simulink model "AGL_FullLoop_DIAM4100"  (R2023a)
settings: Solver=FixedStepAuto  StartTime=0.0  StopTime=DIAM4100.validation.simTime_s  RelTol=1e-3
values from neighbouring files (symbols this model uses):
  DIAM4100 = evalin('base', 'DIAM4100')    [FullLoop_prepareDIAM4100.m]    (also in FullLoop_smokeTest.m)
  FullLoop = evalin('base', 'FullLoop')    [FullLoop_openModel.m]    (also in FullLoop_prepareDIAM4100.m; FullLoop_simParams.m = struct(); FullLoop_smokeTest.m)
undefined symbols (not defined in the file or in its folder): D1, lagging, pulse
libraries: spsSeriesRLCBranchLib x51, spsSaturableTransformerLib x51, spsPiSectionLineLib x50, spsCurrentMeasurementLib x9, spsThyristorLib x2, spsVoltageMeasurementLib x2, spsACVoltageSourceLib x1, slpidlib x1, spsLinearTransformerLib x1, spsPLLLib x1, spsPulseGeneratorThyristor6PulseLib x1, spsRMSLib x1
(part 1 of 2)
settings Model: Creator=KSSS  LastModifiedBy=KSSS

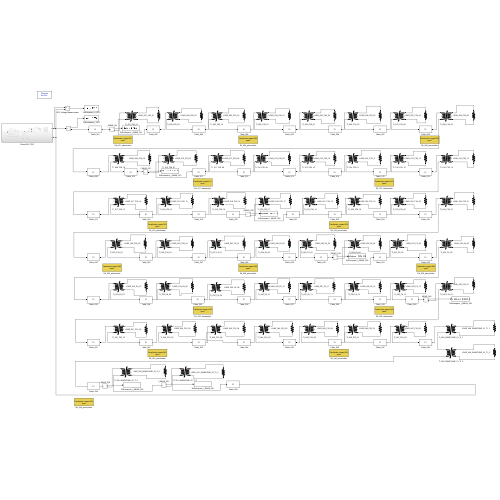
[thumbnail: Simulink's stored preview of the top-level diagram]
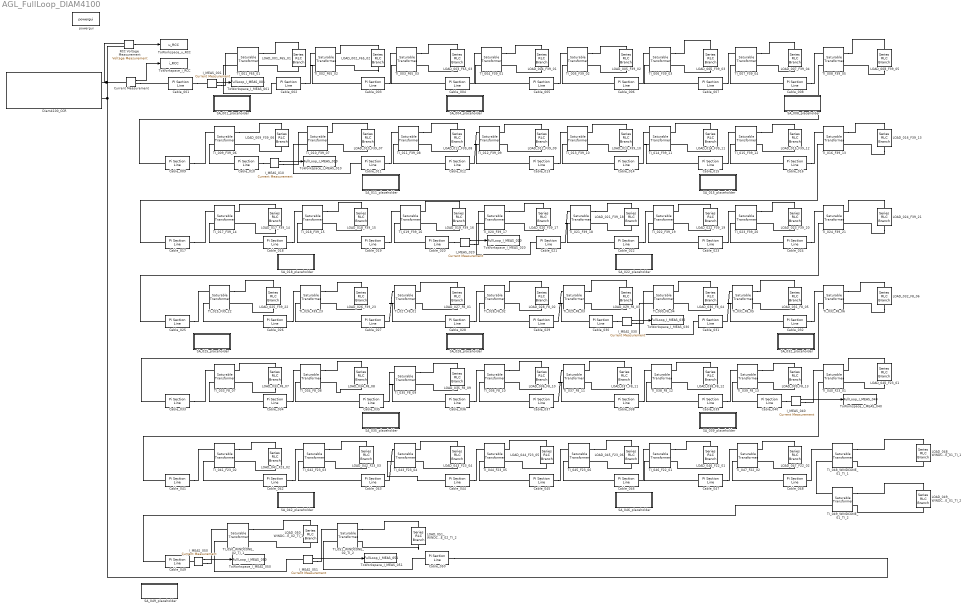
== system AGL_FullLoop_DIAM4100 ==
  Cable_001 : spsPiSectionLineLib/Pi Section Line  LConnTagsString=1  RConnTagsString=1  Phases=1  PiSections=1  Length=FullLoop.segments.length_km(1)  Frequency=FullLoop.grid.f_Hz  Resistance=FullLoop.cable.R_ohm_per_km  Inductance=FullLoop.cable.L_H_per_km  Capacitance=FullLoop.cable.C_F_per_km  SpecifyConductance=off  Conductance=0  Measurements=None  Measurements2=None
      settings: LibrarySourceBlock=sps_lib/Power Grid Elements/Pi Section Line
  Cable_002 : spsPiSectionLineLib/Pi Section Line  LConnTagsString=1  RConnTagsString=1  Phases=1  PiSections=1  Length=FullLoop.segments.length_km(2)  Frequency=FullLoop.grid.f_Hz  Resistance=FullLoop.cable.R_ohm_per_km  Inductance=FullLoop.cable.L_H_per_km  Capacitance=FullLoop.cable.C_F_per_km  SpecifyConductance=off  Conductance=0  Measurements=None  Measurements2=None
      settings: LibrarySourceBlock=sps_lib/Power Grid Elements/Pi Section Line
  Cable_003 : spsPiSectionLineLib/Pi Section Line  LConnTagsString=1  RConnTagsString=1  Phases=1  PiSections=1  Length=FullLoop.segments.length_km(3)  Frequency=FullLoop.grid.f_Hz  Resistance=FullLoop.cable.R_ohm_per_km  Inductance=FullLoop.cable.L_H_per_km  Capacitance=FullLoop.cable.C_F_per_km  SpecifyConductance=off  Conductance=0  Measurements=None  Measurements2=None
      settings: LibrarySourceBlock=sps_lib/Power Grid Elements/Pi Section Line
  Cable_004 : spsPiSectionLineLib/Pi Section Line  LConnTagsString=1  RConnTagsString=1  Phases=1  PiSections=1  Length=FullLoop.segments.length_km(4)  Frequency=FullLoop.grid.f_Hz  Resistance=FullLoop.cable.R_ohm_per_km  Inductance=FullLoop.cable.L_H_per_km  Capacitance=FullLoop.cable.C_F_per_km  SpecifyConductance=off  Conductance=0  Measurements=None  Measurements2=None
      settings: LibrarySourceBlock=sps_lib/Power Grid Elements/Pi Section Line
  Cable_005 : spsPiSectionLineLib/Pi Section Line  LConnTagsString=1  RConnTagsString=1  Phases=1  PiSections=1  Length=FullLoop.segments.length_km(5)  Frequency=FullLoop.grid.f_Hz  Resistance=FullLoop.cable.R_ohm_per_km  Inductance=FullLoop.cable.L_H_per_km  Capacitance=FullLoop.cable.C_F_per_km  SpecifyConductance=off  Conductance=0  Measurements=None  Measurements2=None
      settings: LibrarySourceBlock=sps_lib/Power Grid Elements/Pi Section Line
  Cable_006 : spsPiSectionLineLib/Pi Section Line  LConnTagsString=1  RConnTagsString=1  Phases=1  PiSections=1  Length=FullLoop.segments.length_km(6)  Frequency=FullLoop.grid.f_Hz  Resistance=FullLoop.cable.R_ohm_per_km  Inductance=FullLoop.cable.L_H_per_km  Capacitance=FullLoop.cable.C_F_per_km  SpecifyConductance=off  Conductance=0  Measurements=None  Measurements2=None
      settings: LibrarySourceBlock=sps_lib/Power Grid Elements/Pi Section Line
  Cable_007 : spsPiSectionLineLib/Pi Section Line  LConnTagsString=1  RConnTagsString=1  Phases=1  PiSections=1  Length=FullLoop.segments.length_km(7)  Frequency=FullLoop.grid.f_Hz  Resistance=FullLoop.cable.R_ohm_per_km  Inductance=FullLoop.cable.L_H_per_km  Capacitance=FullLoop.cable.C_F_per_km  SpecifyConductance=off  Conductance=0  Measurements=None  Measurements2=None
      settings: LibrarySourceBlock=sps_lib/Power Grid Elements/Pi Section Line
  Cable_008 : spsPiSectionLineLib/Pi Section Line  LConnTagsString=1  RConnTagsString=1  Phases=1  PiSections=1  Length=FullLoop.segments.length_km(8)  Frequency=FullLoop.grid.f_Hz  Resistance=FullLoop.cable.R_ohm_per_km  Inductance=FullLoop.cable.L_H_per_km  Capacitance=FullLoop.cable.C_F_per_km  SpecifyConductance=off  Conductance=0  Measurements=None  Measurements2=None
      settings: LibrarySourceBlock=sps_lib/Power Grid Elements/Pi Section Line
  Cable_009 : spsPiSectionLineLib/Pi Section Line  LConnTagsString=1  RConnTagsString=1  Phases=1  PiSections=1  Length=FullLoop.segments.length_km(9)  Frequency=FullLoop.grid.f_Hz  Resistance=FullLoop.cable.R_ohm_per_km  Inductance=FullLoop.cable.L_H_per_km  Capacitance=FullLoop.cable.C_F_per_km  SpecifyConductance=off  Conductance=0  Measurements=None  Measurements2=None
      settings: LibrarySourceBlock=sps_lib/Power Grid Elements/Pi Section Line
  Cable_010 : spsPiSectionLineLib/Pi Section Line  LConnTagsString=1  RConnTagsString=1  Phases=1  PiSections=1  Length=FullLoop.segments.length_km(10)  Frequency=FullLoop.grid.f_Hz  Resistance=FullLoop.cable.R_ohm_per_km  Inductance=FullLoop.cable.L_H_per_km  Capacitance=FullLoop.cable.C_F_per_km  SpecifyConductance=off  Conductance=0  Measurements=None  Measurements2=None
      settings: LibrarySourceBlock=sps_lib/Power Grid Elements/Pi Section Line
  Cable_011 : spsPiSectionLineLib/Pi Section Line  LConnTagsString=1  RConnTagsString=1  Phases=1  PiSections=1  Length=FullLoop.segments.length_km(11)  Frequency=FullLoop.grid.f_Hz  Resistance=FullLoop.cable.R_ohm_per_km  Inductance=FullLoop.cable.L_H_per_km  Capacitance=FullLoop.cable.C_F_per_km  SpecifyConductance=off  Conductance=0  Measurements=None  Measurements2=None
      settings: LibrarySourceBlock=sps_lib/Power Grid Elements/Pi Section Line
  Cable_012 : spsPiSectionLineLib/Pi Section Line  LConnTagsString=1  RConnTagsString=1  Phases=1  PiSections=1  Length=FullLoop.segments.length_km(12)  Frequency=FullLoop.grid.f_Hz  Resistance=FullLoop.cable.R_ohm_per_km  Inductance=FullLoop.cable.L_H_per_km  Capacitance=FullLoop.cable.C_F_per_km  SpecifyConductance=off  Conductance=0  Measurements=None  Measurements2=None
      settings: LibrarySourceBlock=sps_lib/Power Grid Elements/Pi Section Line
  Cable_013 : spsPiSectionLineLib/Pi Section Line  LConnTagsString=1  RConnTagsString=1  Phases=1  PiSections=1  Length=FullLoop.segments.length_km(13)  Frequency=FullLoop.grid.f_Hz  Resistance=FullLoop.cable.R_ohm_per_km  Inductance=FullLoop.cable.L_H_per_km  Capacitance=FullLoop.cable.C_F_per_km  SpecifyConductance=off  Conductance=0  Measurements=None  Measurements2=None
      settings: LibrarySourceBlock=sps_lib/Power Grid Elements/Pi Section Line
  Cable_014 : spsPiSectionLineLib/Pi Section Line  LConnTagsString=1  RConnTagsString=1  Phases=1  PiSections=1  Length=FullLoop.segments.length_km(14)  Frequency=FullLoop.grid.f_Hz  Resistance=FullLoop.cable.R_ohm_per_km  Inductance=FullLoop.cable.L_H_per_km  Capacitance=FullLoop.cable.C_F_per_km  SpecifyConductance=off  Conductance=0  Measurements=None  Measurements2=None
      settings: LibrarySourceBlock=sps_lib/Power Grid Elements/Pi Section Line
  Cable_015 : spsPiSectionLineLib/Pi Section Line  LConnTagsString=1  RConnTagsString=1  Phases=1  PiSections=1  Length=FullLoop.segments.length_km(15)  Frequency=FullLoop.grid.f_Hz  Resistance=FullLoop.cable.R_ohm_per_km  Inductance=FullLoop.cable.L_H_per_km  Capacitance=FullLoop.cable.C_F_per_km  SpecifyConductance=off  Conductance=0  Measurements=None  Measurements2=None
      settings: LibrarySourceBlock=sps_lib/Power Grid Elements/Pi Section Line
  Cable_016 : spsPiSectionLineLib/Pi Section Line  LConnTagsString=1  RConnTagsString=1  Phases=1  PiSections=1  Length=FullLoop.segments.length_km(16)  Frequency=FullLoop.grid.f_Hz  Resistance=FullLoop.cable.R_ohm_per_km  Inductance=FullLoop.cable.L_H_per_km  Capacitance=FullLoop.cable.C_F_per_km  SpecifyConductance=off  Conductance=0  Measurements=None  Measurements2=None
      settings: LibrarySourceBlock=sps_lib/Power Grid Elements/Pi Section Line
  Cable_017 : spsPiSectionLineLib/Pi Section Line  LConnTagsString=1  RConnTagsString=1  Phases=1  PiSections=1  Length=FullLoop.segments.length_km(17)  Frequency=FullLoop.grid.f_Hz  Resistance=FullLoop.cable.R_ohm_per_km  Inductance=FullLoop.cable.L_H_per_km  Capacitance=FullLoop.cable.C_F_per_km  SpecifyConductance=off  Conductance=0  Measurements=None  Measurements2=None
      settings: LibrarySourceBlock=sps_lib/Power Grid Elements/Pi Section Line
  Cable_018 : spsPiSectionLineLib/Pi Section Line  LConnTagsString=1  RConnTagsString=1  Phases=1  PiSections=1  Length=FullLoop.segments.length_km(18)  Frequency=FullLoop.grid.f_Hz  Resistance=FullLoop.cable.R_ohm_per_km  Inductance=FullLoop.cable.L_H_per_km  Capacitance=FullLoop.cable.C_F_per_km  SpecifyConductance=off  Conductance=0  Measurements=None  Measurements2=None
      settings: LibrarySourceBlock=sps_lib/Power Grid Elements/Pi Section Line
  Cable_019 : spsPiSectionLineLib/Pi Section Line  LConnTagsString=1  RConnTagsString=1  Phases=1  PiSections=1  Length=FullLoop.segments.length_km(19)  Frequency=FullLoop.grid.f_Hz  Resistance=FullLoop.cable.R_ohm_per_km  Inductance=FullLoop.cable.L_H_per_km  Capacitance=FullLoop.cable.C_F_per_km  SpecifyConductance=off  Conductance=0  Measurements=None  Measurements2=None
      settings: LibrarySourceBlock=sps_lib/Power Grid Elements/Pi Section Line
  Cable_020 : spsPiSectionLineLib/Pi Section Line  LConnTagsString=1  RConnTagsString=1  Phases=1  PiSections=1  Length=FullLoop.segments.length_km(20)  Frequency=FullLoop.grid.f_Hz  Resistance=FullLoop.cable.R_ohm_per_km  Inductance=FullLoop.cable.L_H_per_km  Capacitance=FullLoop.cable.C_F_per_km  SpecifyConductance=off  Conductance=0  Measurements=None  Measurements2=None
      settings: LibrarySourceBlock=sps_lib/Power Grid Elements/Pi Section Line
  Cable_021 : spsPiSectionLineLib/Pi Section Line  LConnTagsString=1  RConnTagsString=1  Phases=1  PiSections=1  Length=FullLoop.segments.length_km(21)  Frequency=FullLoop.grid.f_Hz  Resistance=FullLoop.cable.R_ohm_per_km  Inductance=FullLoop.cable.L_H_per_km  Capacitance=FullLoop.cable.C_F_per_km  SpecifyConductance=off  Conductance=0  Measurements=None  Measurements2=None
      settings: LibrarySourceBlock=sps_lib/Power Grid Elements/Pi Section Line
  Cable_022 : spsPiSectionLineLib/Pi Section Line  LConnTagsString=1  RConnTagsString=1  Phases=1  PiSections=1  Length=FullLoop.segments.length_km(22)  Frequency=FullLoop.grid.f_Hz  Resistance=FullLoop.cable.R_ohm_per_km  Inductance=FullLoop.cable.L_H_per_km  Capacitance=FullLoop.cable.C_F_per_km  SpecifyConductance=off  Conductance=0  Measurements=None  Measurements2=None
      settings: LibrarySourceBlock=sps_lib/Power Grid Elements/Pi Section Line
  Cable_023 : spsPiSectionLineLib/Pi Section Line  LConnTagsString=1  RConnTagsString=1  Phases=1  PiSections=1  Length=FullLoop.segments.length_km(23)  Frequency=FullLoop.grid.f_Hz  Resistance=FullLoop.cable.R_ohm_per_km  Inductance=FullLoop.cable.L_H_per_km  Capacitance=FullLoop.cable.C_F_per_km  SpecifyConductance=off  Conductance=0  Measurements=None  Measurements2=None
      settings: LibrarySourceBlock=sps_lib/Power Grid Elements/Pi Section Line
  Cable_024 : spsPiSectionLineLib/Pi Section Line  LConnTagsString=1  RConnTagsString=1  Phases=1  PiSections=1  Length=FullLoop.segments.length_km(24)  Frequency=FullLoop.grid.f_Hz  Resistance=FullLoop.cable.R_ohm_per_km  Inductance=FullLoop.cable.L_H_per_km  Capacitance=FullLoop.cable.C_F_per_km  SpecifyConductance=off  Conductance=0  Measurements=None  Measurements2=None
      settings: LibrarySourceBlock=sps_lib/Power Grid Elements/Pi Section Line
  Cable_025 : spsPiSectionLineLib/Pi Section Line  LConnTagsString=1  RConnTagsString=1  Phases=1  PiSections=1  Length=FullLoop.segments.length_km(25)  Frequency=FullLoop.grid.f_Hz  Resistance=FullLoop.cable.R_ohm_per_km  Inductance=FullLoop.cable.L_H_per_km  Capacitance=FullLoop.cable.C_F_per_km  SpecifyConductance=off  Conductance=0  Measurements=None  Measurements2=None
      settings: LibrarySourceBlock=sps_lib/Power Grid Elements/Pi Section Line
  Cable_026 : spsPiSectionLineLib/Pi Section Line  LConnTagsString=1  RConnTagsString=1  Phases=1  PiSections=1  Length=FullLoop.segments.length_km(26)  Frequency=FullLoop.grid.f_Hz  Resistance=FullLoop.cable.R_ohm_per_km  Inductance=FullLoop.cable.L_H_per_km  Capacitance=FullLoop.cable.C_F_per_km  SpecifyConductance=off  Conductance=0  Measurements=None  Measurements2=None
      settings: LibrarySourceBlock=sps_lib/Power Grid Elements/Pi Section Line
  Cable_027 : spsPiSectionLineLib/Pi Section Line  LConnTagsString=1  RConnTagsString=1  Phases=1  PiSections=1  Length=FullLoop.segments.length_km(27)  Frequency=FullLoop.grid.f_Hz  Resistance=FullLoop.cable.R_ohm_per_km  Inductance=FullLoop.cable.L_H_per_km  Capacitance=FullLoop.cable.C_F_per_km  SpecifyConductance=off  Conductance=0  Measurements=None  Measurements2=None
      settings: LibrarySourceBlock=sps_lib/Power Grid Elements/Pi Section Line
  Cable_028 : spsPiSectionLineLib/Pi Section Line  LConnTagsString=1  RConnTagsString=1  Phases=1  PiSections=1  Length=FullLoop.segments.length_km(28)  Frequency=FullLoop.grid.f_Hz  Resistance=FullLoop.cable.R_ohm_per_km  Inductance=FullLoop.cable.L_H_per_km  Capacitance=FullLoop.cable.C_F_per_km  SpecifyConductance=off  Conductance=0  Measurements=None  Measurements2=None
      settings: LibrarySourceBlock=sps_lib/Power Grid Elements/Pi Section Line
  Cable_029 : spsPiSectionLineLib/Pi Section Line  LConnTagsString=1  RConnTagsString=1  Phases=1  PiSections=1  Length=FullLoop.segments.length_km(29)  Frequency=FullLoop.grid.f_Hz  Resistance=FullLoop.cable.R_ohm_per_km  Inductance=FullLoop.cable.L_H_per_km  Capacitance=FullLoop.cable.C_F_per_km  SpecifyConductance=off  Conductance=0  Measurements=None  Measurements2=None
      settings: LibrarySourceBlock=sps_lib/Power Grid Elements/Pi Section Line
  Cable_030 : spsPiSectionLineLib/Pi Section Line  LConnTagsString=1  RConnTagsString=1  Phases=1  PiSections=1  Length=FullLoop.segments.length_km(30)  Frequency=FullLoop.grid.f_Hz  Resistance=FullLoop.cable.R_ohm_per_km  Inductance=FullLoop.cable.L_H_per_km  Capacitance=FullLoop.cable.C_F_per_km  SpecifyConductance=off  Conductance=0  Measurements=None  Measurements2=None
      settings: LibrarySourceBlock=sps_lib/Power Grid Elements/Pi Section Line
  Cable_031 : spsPiSectionLineLib/Pi Section Line  LConnTagsString=1  RConnTagsString=1  Phases=1  PiSections=1  Length=FullLoop.segments.length_km(31)  Frequency=FullLoop.grid.f_Hz  Resistance=FullLoop.cable.R_ohm_per_km  Inductance=FullLoop.cable.L_H_per_km  Capacitance=FullLoop.cable.C_F_per_km  SpecifyConductance=off  Conductance=0  Measurements=None  Measurements2=None
      settings: LibrarySourceBlock=sps_lib/Power Grid Elements/Pi Section Line
  Cable_032 : spsPiSectionLineLib/Pi Section Line  LConnTagsString=1  RConnTagsString=1  Phases=1  PiSections=1  Length=FullLoop.segments.length_km(32)  Frequency=FullLoop.grid.f_Hz  Resistance=FullLoop.cable.R_ohm_per_km  Inductance=FullLoop.cable.L_H_per_km  Capacitance=FullLoop.cable.C_F_per_km  SpecifyConductance=off  Conductance=0  Measurements=None  Measurements2=None
      settings: LibrarySourceBlock=sps_lib/Power Grid Elements/Pi Section Line
  Cable_033 : spsPiSectionLineLib/Pi Section Line  LConnTagsString=1  RConnTagsString=1  Phases=1  PiSections=1  Length=FullLoop.segments.length_km(33)  Frequency=FullLoop.grid.f_Hz  Resistance=FullLoop.cable.R_ohm_per_km  Inductance=FullLoop.cable.L_H_per_km  Capacitance=FullLoop.cable.C_F_per_km  SpecifyConductance=off  Conductance=0  Measurements=None  Measurements2=None
      settings: LibrarySourceBlock=sps_lib/Power Grid Elements/Pi Section Line
  Cable_034 : spsPiSectionLineLib/Pi Section Line  LConnTagsString=1  RConnTagsString=1  Phases=1  PiSections=1  Length=FullLoop.segments.length_km(34)  Frequency=FullLoop.grid.f_Hz  Resistance=FullLoop.cable.R_ohm_per_km  Inductance=FullLoop.cable.L_H_per_km  Capacitance=FullLoop.cable.C_F_per_km  SpecifyConductance=off  Conductance=0  Measurements=None  Measurements2=None
      settings: LibrarySourceBlock=sps_lib/Power Grid Elements/Pi Section Line
  Cable_035 : spsPiSectionLineLib/Pi Section Line  LConnTagsString=1  RConnTagsString=1  Phases=1  PiSections=1  Length=FullLoop.segments.length_km(35)  Frequency=FullLoop.grid.f_Hz  Resistance=FullLoop.cable.R_ohm_per_km  Inductance=FullLoop.cable.L_H_per_km  Capacitance=FullLoop.cable.C_F_per_km  SpecifyConductance=off  Conductance=0  Measurements=None  Measurements2=None
      settings: LibrarySourceBlock=sps_lib/Power Grid Elements/Pi Section Line
  Cable_036 : spsPiSectionLineLib/Pi Section Line  LConnTagsString=1  RConnTagsString=1  Phases=1  PiSections=1  Length=FullLoop.segments.length_km(36)  Frequency=FullLoop.grid.f_Hz  Resistance=FullLoop.cable.R_ohm_per_km  Inductance=FullLoop.cable.L_H_per_km  Capacitance=FullLoop.cable.C_F_per_km  SpecifyConductance=off  Conductance=0  Measurements=None  Measurements2=None
      settings: LibrarySourceBlock=sps_lib/Power Grid Elements/Pi Section Line
  Cable_037 : spsPiSectionLineLib/Pi Section Line  LConnTagsString=1  RConnTagsString=1  Phases=1  PiSections=1  Length=FullLoop.segments.length_km(37)  Frequency=FullLoop.grid.f_Hz  Resistance=FullLoop.cable.R_ohm_per_km  Inductance=FullLoop.cable.L_H_per_km  Capacitance=FullLoop.cable.C_F_per_km  SpecifyConductance=off  Conductance=0  Measurements=None  Measurements2=None
      settings: LibrarySourceBlock=sps_lib/Power Grid Elements/Pi Section Line
  Cable_038 : spsPiSectionLineLib/Pi Section Line  LConnTagsString=1  RConnTagsString=1  Phases=1  PiSections=1  Length=FullLoop.segments.length_km(38)  Frequency=FullLoop.grid.f_Hz  Resistance=FullLoop.cable.R_ohm_per_km  Inductance=FullLoop.cable.L_H_per_km  Capacitance=FullLoop.cable.C_F_per_km  SpecifyConductance=off  Conductance=0  Measurements=None  Measurements2=None
      settings: LibrarySourceBlock=sps_lib/Power Grid Elements/Pi Section Line
  Cable_039 : spsPiSectionLineLib/Pi Section Line  LConnTagsString=1  RConnTagsString=1  Phases=1  PiSections=1  Length=FullLoop.segments.length_km(39)  Frequency=FullLoop.grid.f_Hz  Resistance=FullLoop.cable.R_ohm_per_km  Inductance=FullLoop.cable.L_H_per_km  Capacitance=FullLoop.cable.C_F_per_km  SpecifyConductance=off  Conductance=0  Measurements=None  Measurements2=None
      settings: LibrarySourceBlock=sps_lib/Power Grid Elements/Pi Section Line
  Cable_040 : spsPiSectionLineLib/Pi Section Line  LConnTagsString=1  RConnTagsString=1  Phases=1  PiSections=1  Length=FullLoop.segments.length_km(40)  Frequency=FullLoop.grid.f_Hz  Resistance=FullLoop.cable.R_ohm_per_km  Inductance=FullLoop.cable.L_H_per_km  Capacitance=FullLoop.cable.C_F_per_km  SpecifyConductance=off  Conductance=0  Measurements=None  Measurements2=None
      settings: LibrarySourceBlock=sps_lib/Power Grid Elements/Pi Section Line
  Cable_041 : spsPiSectionLineLib/Pi Section Line  LConnTagsString=1  RConnTagsString=1  Phases=1  PiSections=1  Length=FullLoop.segments.length_km(41)  Frequency=FullLoop.grid.f_Hz  Resistance=FullLoop.cable.R_ohm_per_km  Inductance=FullLoop.cable.L_H_per_km  Capacitance=FullLoop.cable.C_F_per_km  SpecifyConductance=off  Conductance=0  Measurements=None  Measurements2=None
      settings: LibrarySourceBlock=sps_lib/Power Grid Elements/Pi Section Line
  Cable_042 : spsPiSectionLineLib/Pi Section Line  LConnTagsString=1  RConnTagsString=1  Phases=1  PiSections=1  Length=FullLoop.segments.length_km(42)  Frequency=FullLoop.grid.f_Hz  Resistance=FullLoop.cable.R_ohm_per_km  Inductance=FullLoop.cable.L_H_per_km  Capacitance=FullLoop.cable.C_F_per_km  SpecifyConductance=off  Conductance=0  Measurements=None  Measurements2=None
      settings: LibrarySourceBlock=sps_lib/Power Grid Elements/Pi Section Line
  Cable_043 : spsPiSectionLineLib/Pi Section Line  LConnTagsString=1  RConnTagsString=1  Phases=1  PiSections=1  Length=FullLoop.segments.length_km(43)  Frequency=FullLoop.grid.f_Hz  Resistance=FullLoop.cable.R_ohm_per_km  Inductance=FullLoop.cable.L_H_per_km  Capacitance=FullLoop.cable.C_F_per_km  SpecifyConductance=off  Conductance=0  Measurements=None  Measurements2=None
      settings: LibrarySourceBlock=sps_lib/Power Grid Elements/Pi Section Line
  Cable_044 : spsPiSectionLineLib/Pi Section Line  LConnTagsString=1  RConnTagsString=1  Phases=1  PiSections=1  Length=FullLoop.segments.length_km(44)  Frequency=FullLoop.grid.f_Hz  Resistance=FullLoop.cable.R_ohm_per_km  Inductance=FullLoop.cable.L_H_per_km  Capacitance=FullLoop.cable.C_F_per_km  SpecifyConductance=off  Conductance=0  Measurements=None  Measurements2=None
      settings: LibrarySourceBlock=sps_lib/Power Grid Elements/Pi Section Line
  Cable_045 : spsPiSectionLineLib/Pi Section Line  LConnTagsString=1  RConnTagsString=1  Phases=1  PiSections=1  Length=FullLoop.segments.length_km(45)  Frequency=FullLoop.grid.f_Hz  Resistance=FullLoop.cable.R_ohm_per_km  Inductance=FullLoop.cable.L_H_per_km  Capacitance=FullLoop.cable.C_F_per_km  SpecifyConductance=off  Conductance=0  Measurements=None  Measurements2=None
      settings: LibrarySourceBlock=sps_lib/Power Grid Elements/Pi Section Line
  Cable_046 : spsPiSectionLineLib/Pi Section Line  LConnTagsString=1  RConnTagsString=1  Phases=1  PiSections=1  Length=FullLoop.segments.length_km(46)  Frequency=FullLoop.grid.f_Hz  Resistance=FullLoop.cable.R_ohm_per_km  Inductance=FullLoop.cable.L_H_per_km  Capacitance=FullLoop.cable.C_F_per_km  SpecifyConductance=off  Conductance=0  Measurements=None  Measurements2=None
      settings: LibrarySourceBlock=sps_lib/Power Grid Elements/Pi Section Line
  Cable_047 : spsPiSectionLineLib/Pi Section Line  LConnTagsString=1  RConnTagsString=1  Phases=1  PiSections=1  Length=FullLoop.segments.length_km(47)  Frequency=FullLoop.grid.f_Hz  Resistance=FullLoop.cable.R_ohm_per_km  Inductance=FullLoop.cable.L_H_per_km  Capacitance=FullLoop.cable.C_F_per_km  SpecifyConductance=off  Conductance=0  Measurements=None  Measurements2=None
      settings: LibrarySourceBlock=sps_lib/Power Grid Elements/Pi Section Line
  Cable_048 : spsPiSectionLineLib/Pi Section Line  LConnTagsString=1  RConnTagsString=1  Phases=1  PiSections=1  Length=FullLoop.segments.length_km(48)  Frequency=FullLoop.grid.f_Hz  Resistance=FullLoop.cable.R_ohm_per_km  Inductance=FullLoop.cable.L_H_per_km  Capacitance=FullLoop.cable.C_F_per_km  SpecifyConductance=off  Conductance=0  Measurements=None  Measurements2=None
      settings: LibrarySourceBlock=sps_lib/Power Grid Elements/Pi Section Line
  Cable_049 : spsPiSectionLineLib/Pi Section Line  LConnTagsString=1  RConnTagsString=1  Phases=1  PiSections=1  Length=FullLoop.segments.length_km(49)  Frequency=FullLoop.grid.f_Hz  Resistance=FullLoop.cable.R_ohm_per_km  Inductance=FullLoop.cable.L_H_per_km  Capacitance=FullLoop.cable.C_F_per_km  SpecifyConductance=off  Conductance=0  Measurements=None  Measurements2=None
      settings: LibrarySourceBlock=sps_lib/Power Grid Elements/Pi Section Line
  Cable_050 : spsPiSectionLineLib/Pi Section Line  LConnTagsString=1  RConnTagsString=1  Phases=1  PiSections=1  Length=FullLoop.segments.length_km(50)  Frequency=FullLoop.grid.f_Hz  Resistance=FullLoop.cable.R_ohm_per_km  Inductance=FullLoop.cable.L_H_per_km  Capacitance=FullLoop.cable.C_F_per_km  SpecifyConductance=off  Conductance=0  Measurements=None  Measurements2=None
      settings: LibrarySourceBlock=sps_lib/Power Grid Elements/Pi Section Line
  Current Measurement : spsCurrentMeasurementLib/Current Measurement  PhasorSimulation=off  OutputType=Complex  PSBequivalent=0
  Diam4100_CCR : Subsystem
  I_MEAS_001 : spsCurrentMeasurementLib/Current Measurement  PhasorSimulation=off  OutputType=Complex  PSBequivalent=0
  I_MEAS_010 : spsCurrentMeasurementLib/Current Measurement  PhasorSimulation=off  OutputType=Complex  PSBequivalent=0
  I_MEAS_020 : spsCurrentMeasurementLib/Current Measurement  PhasorSimulation=off  OutputType=Complex  PSBequivalent=0
  I_MEAS_030 : spsCurrentMeasurementLib/Current Measurement  PhasorSimulation=off  OutputType=Complex  PSBequivalent=0
  I_MEAS_040 : spsCurrentMeasurementLib/Current Measurement  PhasorSimulation=off  OutputType=Complex  PSBequivalent=0
  I_MEAS_050 : spsCurrentMeasurementLib/Current Measurement  PhasorSimulation=off  OutputType=Complex  PSBequivalent=0
  I_MEAS_051 : spsCurrentMeasurementLib/Current Measurement  PhasorSimulation=off  OutputType=Complex  PSBequivalent=0
  LOAD_001_F65_01 : spsSeriesRLCBranchLib/Series RLC Branch  LConnTagsString=__new0  RConnTagsString=__new0  BranchType=R  Resistance=FullLoop.loads(1).SecondaryResistance_ohm  Inductance=1e-3  SetiL0=off  InitialCurrent=0  Capacitance=1e-6  Setx0=off  InitialVoltage=0  Measurements=None
  LOAD_002_F65_02 : spsSeriesRLCBranchLib/Series RLC Branch  LConnTagsString=__new0  RConnTagsString=__new0  BranchType=R  Resistance=FullLoop.loads(2).SecondaryResistance_ohm  Inductance=1e-3  SetiL0=off  InitialCurrent=0  Capacitance=1e-6  Setx0=off  InitialVoltage=0  Measurements=None
  LOAD_003_F65_03 : spsSeriesRLCBranchLib/Series RLC Branch  LConnTagsString=__new0  RConnTagsString=__new0  BranchType=R  Resistance=FullLoop.loads(3).SecondaryResistance_ohm  Inductance=1e-3  SetiL0=off  InitialCurrent=0  Capacitance=1e-6  Setx0=off  InitialVoltage=0  Measurements=None
  LOAD_004_F39_01 : spsSeriesRLCBranchLib/Series RLC Branch  LConnTagsString=__new0  RConnTagsString=__new0  BranchType=R  Resistance=FullLoop.loads(4).SecondaryResistance_ohm  Inductance=1e-3  SetiL0=off  InitialCurrent=0  Capacitance=1e-6  Setx0=off  InitialVoltage=0  Measurements=None
  LOAD_005_F39_02 : spsSeriesRLCBranchLib/Series RLC Branch  LConnTagsString=__new0  RConnTagsString=__new0  BranchType=R  Resistance=FullLoop.loads(5).SecondaryResistance_ohm  Inductance=1e-3  SetiL0=off  InitialCurrent=0  Capacitance=1e-6  Setx0=off  InitialVoltage=0  Measurements=None
  LOAD_006_F39_03 : spsSeriesRLCBranchLib/Series RLC Branch  LConnTagsString=__new0  RConnTagsString=__new0  BranchType=R  Resistance=FullLoop.loads(6).SecondaryResistance_ohm  Inductance=1e-3  SetiL0=off  InitialCurrent=0  Capacitance=1e-6  Setx0=off  InitialVoltage=0  Measurements=None
  LOAD_007_F39_04 : spsSeriesRLCBranchLib/Series RLC Branch  LConnTagsString=__new0  RConnTagsString=__new0  BranchType=R  Resistance=FullLoop.loads(7).SecondaryResistance_ohm  Inductance=1e-3  SetiL0=off  InitialCurrent=0  Capacitance=1e-6  Setx0=off  InitialVoltage=0  Measurements=None
  LOAD_008_F39_05 : spsSeriesRLCBranchLib/Series RLC Branch  LConnTagsString=__new0  RConnTagsString=__new0  BranchType=R  Resistance=FullLoop.loads(8).SecondaryResistance_ohm  Inductance=1e-3  SetiL0=off  InitialCurrent=0  Capacitance=1e-6  Setx0=off  InitialVoltage=0  Measurements=None
  LOAD_009_F39_06 : spsSeriesRLCBranchLib/Series RLC Branch  LConnTagsString=__new0  RConnTagsString=__new0  BranchType=R  Resistance=FullLoop.loads(9).SecondaryResistance_ohm  Inductance=1e-3  SetiL0=off  InitialCurrent=0  Capacitance=1e-6  Setx0=off  InitialVoltage=0  Measurements=None
  LOAD_010_F39_07 : spsSeriesRLCBranchLib/Series RLC Branch  LConnTagsString=__new0  RConnTagsString=__new0  BranchType=R  Resistance=FullLoop.loads(10).SecondaryResistance_ohm  Inductance=1e-3  SetiL0=off  InitialCurrent=0  Capacitance=1e-6  Setx0=off  InitialVoltage=0  Measurements=None
  LOAD_011_F39_08 : spsSeriesRLCBranchLib/Series RLC Branch  LConnTagsString=__new0  RConnTagsString=__new0  BranchType=R  Resistance=FullLoop.loads(11).SecondaryResistance_ohm  Inductance=1e-3  SetiL0=off  InitialCurrent=0  Capacitance=1e-6  Setx0=off  InitialVoltage=0  Measurements=None
  LOAD_012_F39_09 : spsSeriesRLCBranchLib/Series RLC Branch  LConnTagsString=__new0  RConnTagsString=__new0  BranchType=R  Resistance=FullLoop.loads(12).SecondaryResistance_ohm  Inductance=1e-3  SetiL0=off  InitialCurrent=0  Capacitance=1e-6  Setx0=off  InitialVoltage=0  Measurements=None
  LOAD_013_F39_10 : spsSeriesRLCBranchLib/Series RLC Branch  LConnTagsString=__new0  RConnTagsString=__new0  BranchType=R  Resistance=FullLoop.loads(13).SecondaryResistance_ohm  Inductance=1e-3  SetiL0=off  InitialCurrent=0  Capacitance=1e-6  Setx0=off  InitialVoltage=0  Measurements=None
  LOAD_014_F39_11 : spsSeriesRLCBranchLib/Series RLC Branch  LConnTagsString=__new0  RConnTagsString=__new0  BranchType=R  Resistance=FullLoop.loads(14).SecondaryResistance_ohm  Inductance=1e-3  SetiL0=off  InitialCurrent=0  Capacitance=1e-6  Setx0=off  InitialVoltage=0  Measurements=None
  LOAD_015_F39_12 : spsSeriesRLCBranchLib/Series RLC Branch  LConnTagsString=__new0  RConnTagsString=__new0  BranchType=R  Resistance=FullLoop.loads(15).SecondaryResistance_ohm  Inductance=1e-3  SetiL0=off  InitialCurrent=0  Capacitance=1e-6  Setx0=off  InitialVoltage=0  Measurements=None
  LOAD_016_F39_13 : spsSeriesRLCBranchLib/Series RLC Branch  LConnTagsString=__new0  RConnTagsString=__new0  BranchType=R  Resistance=FullLoop.loads(16).SecondaryResistance_ohm  Inductance=1e-3  SetiL0=off  InitialCurrent=0  Capacitance=1e-6  Setx0=off  InitialVoltage=0  Measurements=None
  LOAD_017_F39_14 : spsSeriesRLCBranchLib/Series RLC Branch  LConnTagsString=__new0  RConnTagsString=__new0  BranchType=R  Resistance=FullLoop.loads(17).SecondaryResistance_ohm  Inductance=1e-3  SetiL0=off  InitialCurrent=0  Capacitance=1e-6  Setx0=off  InitialVoltage=0  Measurements=None
  LOAD_018_F39_15 : spsSeriesRLCBranchLib/Series RLC Branch  LConnTagsString=__new0  RConnTagsString=__new0  BranchType=R  Resistance=FullLoop.loads(18).SecondaryResistance_ohm  Inductance=1e-3  SetiL0=off  InitialCurrent=0  Capacitance=1e-6  Setx0=off  InitialVoltage=0  Measurements=None
  LOAD_019_F39_16 : spsSeriesRLCBranchLib/Series RLC Branch  LConnTagsString=__new0  RConnTagsString=__new0  BranchType=R  Resistance=FullLoop.loads(19).SecondaryResistance_ohm  Inductance=1e-3  SetiL0=off  InitialCurrent=0  Capacitance=1e-6  Setx0=off  InitialVoltage=0  Measurements=None
  LOAD_020_F39_17 : spsSeriesRLCBranchLib/Series RLC Branch  LConnTagsString=__new0  RConnTagsString=__new0  BranchType=R  Resistance=FullLoop.loads(20).SecondaryResistance_ohm  Inductance=1e-3  SetiL0=off  InitialCurrent=0  Capacitance=1e-6  Setx0=off  InitialVoltage=0  Measurements=None
  LOAD_021_F39_18 : spsSeriesRLCBranchLib/Series RLC Branch  LConnTagsString=__new0  RConnTagsString=__new0  BranchType=R  Resistance=FullLoop.loads(21).SecondaryResistance_ohm  Inductance=1e-3  SetiL0=off  InitialCurrent=0  Capacitance=1e-6  Setx0=off  InitialVoltage=0  Measurements=None
  LOAD_022_F39_19 : spsSeriesRLCBranchLib/Series RLC Branch  LConnTagsString=__new0  RConnTagsString=__new0  BranchType=R  Resistance=FullLoop.loads(22).SecondaryResistance_ohm  Inductance=1e-3  SetiL0=off  InitialCurrent=0  Capacitance=1e-6  Setx0=off  InitialVoltage=0  Measurements=None
  LOAD_023_F39_20 : spsSeriesRLCBranchLib/Series RLC Branch  LConnTagsString=__new0  RConnTagsString=__new0  BranchType=R  Resistance=FullLoop.loads(23).SecondaryResistance_ohm  Inductance=1e-3  SetiL0=off  InitialCurrent=0  Capacitance=1e-6  Setx0=off  InitialVoltage=0  Measurements=None
  LOAD_024_F39_21 : spsSeriesRLCBranchLib/Series RLC Branch  LConnTagsString=__new0  RConnTagsString=__new0  BranchType=R  Resistance=FullLoop.loads(24).SecondaryResistance_ohm  Inductance=1e-3  SetiL0=off  InitialCurrent=0  Capacitance=1e-6  Setx0=off  InitialVoltage=0  Measurements=None
  LOAD_025_F39_22 : spsSeriesRLCBranchLib/Series RLC Branch  LConnTagsString=__new0  RConnTagsString=__new0  BranchType=R  Resistance=FullLoop.loads(25).SecondaryResistance_ohm  Inductance=1e-3  SetiL0=off  InitialCurrent=0  Capacitance=1e-6  Setx0=off  InitialVoltage=0  Measurements=None
  LOAD_026_F39_23 : spsSeriesRLCBranchLib/Series RLC Branch  LConnTagsString=__new0  RConnTagsString=__new0  BranchType=R  Resistance=FullLoop.loads(26).SecondaryResistance_ohm  Inductance=1e-3  SetiL0=off  InitialCurrent=0  Capacitance=1e-6  Setx0=off  InitialVoltage=0  Measurements=None
  LOAD_027_F8_01 : spsSeriesRLCBranchLib/Series RLC Branch  LConnTagsString=__new0  RConnTagsString=__new0  BranchType=R  Resistance=FullLoop.loads(27).SecondaryResistance_ohm  Inductance=1e-3  SetiL0=off  InitialCurrent=0  Capacitance=1e-6  Setx0=off  InitialVoltage=0  Measurements=None
  LOAD_028_F8_02 : spsSeriesRLCBranchLib/Series RLC Branch  LConnTagsString=__new0  RConnTagsString=__new0  BranchType=R  Resistance=FullLoop.loads(28).SecondaryResistance_ohm  Inductance=1e-3  SetiL0=off  InitialCurrent=0  Capacitance=1e-6  Setx0=off  InitialVoltage=0  Measurements=None
  LOAD_029_F8_03 : spsSeriesRLCBranchLib/Series RLC Branch  LConnTagsString=__new0  RConnTagsString=__new0  BranchType=R  Resistance=FullLoop.loads(29).SecondaryResistance_ohm  Inductance=1e-3  SetiL0=off  InitialCurrent=0  Capacitance=1e-6  Setx0=off  InitialVoltage=0  Measurements=None
  LOAD_030_F8_04 : spsSeriesRLCBranchLib/Series RLC Branch  LConnTagsString=__new0  RConnTagsString=__new0  BranchType=R  Resistance=FullLoop.loads(30).SecondaryResistance_ohm  Inductance=1e-3  SetiL0=off  InitialCurrent=0  Capacitance=1e-6  Setx0=off  InitialVoltage=0  Measurements=None
  LOAD_031_F8_05 : spsSeriesRLCBranchLib/Series RLC Branch  LConnTagsString=__new0  RConnTagsString=__new0  BranchType=R  Resistance=FullLoop.loads(31).SecondaryResistance_ohm  Inductance=1e-3  SetiL0=off  InitialCurrent=0  Capacitance=1e-6  Setx0=off  InitialVoltage=0  Measurements=None
  LOAD_032_F8_06 : spsSeriesRLCBranchLib/Series RLC Branch  LConnTagsString=__new0  RConnTagsString=__new0  BranchType=R  Resistance=FullLoop.loads(32).SecondaryResistance_ohm  Inductance=1e-3  SetiL0=off  InitialCurrent=0  Capacitance=1e-6  Setx0=off  InitialVoltage=0  Measurements=None
  LOAD_033_F8_07 : spsSeriesRLCBranchLib/Series RLC Branch  LConnTagsString=__new0  RConnTagsString=__new0  BranchType=R  Resistance=FullLoop.loads(33).SecondaryResistance_ohm  Inductance=1e-3  SetiL0=off  InitialCurrent=0  Capacitance=1e-6  Setx0=off  InitialVoltage=0  Measurements=None
  LOAD_034_F8_08 : spsSeriesRLCBranchLib/Series RLC Branch  LConnTagsString=__new0  RConnTagsString=__new0  BranchType=R  Resistance=FullLoop.loads(34).SecondaryResistance_ohm  Inductance=1e-3  SetiL0=off  InitialCurrent=0  Capacitance=1e-6  Setx0=off  InitialVoltage=0  Measurements=None
  LOAD_035_F8_09 : spsSeriesRLCBranchLib/Series RLC Branch  LConnTagsString=__new0  RConnTagsString=__new0  BranchType=R  Resistance=FullLoop.loads(35).SecondaryResistance_ohm  Inductance=1e-3  SetiL0=off  InitialCurrent=0  Capacitance=1e-6  Setx0=off  InitialVoltage=0  Measurements=None
  LOAD_036_F8_10 : spsSeriesRLCBranchLib/Series RLC Branch  LConnTagsString=__new0  RConnTagsString=__new0  BranchType=R  Resistance=FullLoop.loads(36).SecondaryResistance_ohm  Inductance=1e-3  SetiL0=off  InitialCurrent=0  Capacitance=1e-6  Setx0=off  InitialVoltage=0  Measurements=None
  LOAD_037_F8_11 : spsSeriesRLCBranchLib/Series RLC Branch  LConnTagsString=__new0  RConnTagsString=__new0  BranchType=R  Resistance=FullLoop.loads(37).SecondaryResistance_ohm  Inductance=1e-3  SetiL0=off  InitialCurrent=0  Capacitance=1e-6  Setx0=off  InitialVoltage=0  Measurements=None
  LOAD_038_F8_12 : spsSeriesRLCBranchLib/Series RLC Branch  LConnTagsString=__new0  RConnTagsString=__new0  BranchType=R  Resistance=FullLoop.loads(38).SecondaryResistance_ohm  Inductance=1e-3  SetiL0=off  InitialCurrent=0  Capacitance=1e-6  Setx0=off  InitialVoltage=0  Measurements=None
  LOAD_039_F8_13 : spsSeriesRLCBranchLib/Series RLC Branch  LConnTagsString=__new0  RConnTagsString=__new0  BranchType=R  Resistance=FullLoop.loads(39).SecondaryResistance_ohm  Inductance=1e-3  SetiL0=off  InitialCurrent=0  Capacitance=1e-6  Setx0=off  InitialVoltage=0  Measurements=None
  LOAD_040_F23_01 : spsSeriesRLCBranchLib/Series RLC Branch  LConnTagsString=__new0  RConnTagsString=__new0  BranchType=R  Resistance=FullLoop.loads(40).SecondaryResistance_ohm  Inductance=1e-3  SetiL0=off  InitialCurrent=0  Capacitance=1e-6  Setx0=off  InitialVoltage=0  Measurements=None
  LOAD_041_F23_02 : spsSeriesRLCBranchLib/Series RLC Branch  LConnTagsString=__new0  RConnTagsString=__new0  BranchType=R  Resistance=FullLoop.loads(41).SecondaryResistance_ohm  Inductance=1e-3  SetiL0=off  InitialCurrent=0  Capacitance=1e-6  Setx0=off  InitialVoltage=0  Measurements=None
  LOAD_042_F23_03 : spsSeriesRLCBranchLib/Series RLC Branch  LConnTagsString=__new0  RConnTagsString=__new0  BranchType=R  Resistance=FullLoop.loads(42).SecondaryResistance_ohm  Inductance=1e-3  SetiL0=off  InitialCurrent=0  Capacitance=1e-6  Setx0=off  InitialVoltage=0  Measurements=None
  LOAD_043_F23_04 : spsSeriesRLCBranchLib/Series RLC Branch  LConnTagsString=__new0  RConnTagsString=__new0  BranchType=R  Resistance=FullLoop.loads(43).SecondaryResistance_ohm  Inductance=1e-3  SetiL0=off  InitialCurrent=0  Capacitance=1e-6  Setx0=off  InitialVoltage=0  Measurements=None
  LOAD_044_F23_05 : spsSeriesRLCBranchLib/Series RLC Branch  LConnTagsString=__new0  RConnTagsString=__new0  BranchType=R  Resistance=FullLoop.loads(44).SecondaryResistance_ohm  Inductance=1e-3  SetiL0=off  InitialCurrent=0  Capacitance=1e-6  Setx0=off  InitialVoltage=0  Measurements=None
  LOAD_045_F23_06 : spsSeriesRLCBranchLib/Series RLC Branch  LConnTagsString=__new0  RConnTagsString=__new0  BranchType=R  Resistance=FullLoop.loads(45).SecondaryResistance_ohm  Inductance=1e-3  SetiL0=off  InitialCurrent=0  Capacitance=1e-6  Setx0=off  InitialVoltage=0  Measurements=None
  LOAD_046_F22_01 : spsSeriesRLCBranchLib/Series RLC Branch  LConnTagsString=__new0  RConnTagsString=__new0  BranchType=R  Resistance=FullLoop.loads(46).SecondaryResistance_ohm  Inductance=1e-3  SetiL0=off  InitialCurrent=0  Capacitance=1e-6  Setx0=off  InitialVoltage=0  Measurements=None
  LOAD_047_F22_02 : spsSeriesRLCBranchLib/Series RLC Branch  LConnTagsString=__new0  RConnTagsString=__new0  BranchType=R  Resistance=FullLoop.loads(47).SecondaryResistance_ohm  Inductance=1e-3  SetiL0=off  InitialCurrent=0  Capacitance=1e-6  Setx0=off  InitialVoltage=0  Measurements=None
  LOAD_048_WINDCONE_01_TI_1 : spsSeriesRLCBranchLib/Series RLC Branch  LConnTagsString=__new0  RConnTagsString=__new0  BranchType=R  Resistance=FullLoop.loads(48).SecondaryResistance_ohm  Inductance=1e-3  SetiL0=off  InitialCurrent=0  Capacitance=1e-6  Setx0=off  InitialVoltage=0  Measurements=None
  LOAD_049_WINDCONE_01_TI_2 : spsSeriesRLCBranchLib/Series RLC Branch  LConnTagsString=__new0  RConnTagsString=__new0  BranchType=R  Resistance=FullLoop.loads(49).SecondaryResistance_ohm  Inductance=1e-3  SetiL0=off  InitialCurrent=0  Capacitance=1e-6  Setx0=off  InitialVoltage=0  Measurements=None
  LOAD_050_WINDCONE_02_TI_1 : spsSeriesRLCBranchLib/Series RLC Branch  LConnTagsString=__new0  RConnTagsString=__new0  BranchType=R  Resistance=FullLoop.loads(50).SecondaryResistance_ohm  Inductance=1e-3  SetiL0=off  InitialCurrent=0  Capacitance=1e-6  Setx0=off  InitialVoltage=0  Measurements=None
  LOAD_051_WINDCONE_02_TI_2 : spsSeriesRLCBranchLib/Series RLC Branch  LConnTagsString=__new0  RConnTagsString=__new0  BranchType=R  Resistance=FullLoop.loads(51).SecondaryResistance_ohm  Inductance=1e-3  SetiL0=off  InitialCurrent=0  Capacitance=1e-6  Setx0=off  InitialVoltage=0  Measurements=None
  RCC Voltage Measurement : spsVoltageMeasurementLib/Voltage Measurement  PhasorSimulation=off  OutputType=Complex  PSBequivalent=0
  SA_001_placeholder : Subsystem
      mask Display: disp('Parafoudre regard 001\nopen')
  SA_004_placeholder : Subsystem
      mask Display: disp('Parafoudre regard 004\nopen')
  SA_008_placeholder : Subsystem
      mask Display: disp('Parafoudre regard 008\nopen')
  SA_011_placeholder : Subsystem
      mask Display: disp('Parafoudre regard 011\nopen')
  SA_015_placeholder : Subsystem
      mask Display: disp('Parafoudre regard 015\nopen')
  SA_018_placeholder : Subsystem
      mask Display: disp('Parafoudre regard 018\nopen')
  SA_022_placeholder : Subsystem
      mask Display: disp('Parafoudre regard 022\nopen')
  SA_025_placeholder : Subsystem
      mask Display: disp('Parafoudre regard 025\nopen')
  SA_028_placeholder : Subsystem
      mask Display: disp('Parafoudre regard 028\nopen')
  SA_032_placeholder : Subsystem
      mask Display: disp('Parafoudre regard 032\nopen')
  SA_035_placeholder : Subsystem
      mask Display: disp('Parafoudre regard 035\nopen')
  SA_039_placeholder : Subsystem
      mask Display: disp('Parafoudre regard 039\nopen')
  SA_042_placeholder : Subsystem
      mask Display: disp('Parafoudre regard 042\nopen')
  SA_046_placeholder : Subsystem
      mask Display: disp('Parafoudre regard 046\nopen')
  SA_049_placeholder : Subsystem
      mask Display: disp('Parafoudre regard 049\nopen')
  TI_001_F65_01 : spsSaturableTransformerLib/Saturable Transformer  ThreeWindings=off  Hysteresis=off  DataFile='hysteresis.mat'  Measurements=None  UNITS=SI  NominalPower=FullLoop.tiModules(1).Pn_fn  Winding1=FullLoop.tiModules(1).W1  Winding2=FullLoop.tiModules(1).W2  Winding3=[3.15e+05 1.2118e+09 4.0926e+05]  Saturation=FullLoop.tiModules(1).Sat  CoreLoss=TI_OCEM.Rm  BreakLoop=off  DiscreteSolver=Trapezoidal iterative  DataType=on  InitialFlux=0.0205600583592649  TransfoNumber=1
      settings: LibrarySourceBlock=sps_lib/Power Grid Elements/Saturable Transformer
  TI_002_F65_02 : spsSaturableTransformerLib/Saturable Transformer  ThreeWindings=off  Hysteresis=off  DataFile='hysteresis.mat'  Measurements=None  UNITS=SI  NominalPower=FullLoop.tiModules(2).Pn_fn  Winding1=FullLoop.tiModules(2).W1  Winding2=FullLoop.tiModules(2).W2  Winding3=[3.15e+05 1.2118e+09 4.0926e+05]  Saturation=FullLoop.tiModules(2).Sat  CoreLoss=TI_OCEM.Rm  BreakLoop=off  DiscreteSolver=Trapezoidal iterative  DataType=on  InitialFlux=0.0205600583592649  TransfoNumber=1
      settings: LibrarySourceBlock=sps_lib/Power Grid Elements/Saturable Transformer
  TI_003_F65_03 : spsSaturableTransformerLib/Saturable Transformer  ThreeWindings=off  Hysteresis=off  DataFile='hysteresis.mat'  Measurements=None  UNITS=SI  NominalPower=FullLoop.tiModules(3).Pn_fn  Winding1=FullLoop.tiModules(3).W1  Winding2=FullLoop.tiModules(3).W2  Winding3=[3.15e+05 1.2118e+09 4.0926e+05]  Saturation=FullLoop.tiModules(3).Sat  CoreLoss=TI_OCEM.Rm  BreakLoop=off  DiscreteSolver=Trapezoidal iterative  DataType=on  InitialFlux=0.0205600583592649  TransfoNumber=1
      settings: LibrarySourceBlock=sps_lib/Power Grid Elements/Saturable Transformer
  TI_004_F39_01 : spsSaturableTransformerLib/Saturable Transformer  ThreeWindings=off  Hysteresis=off  DataFile='hysteresis.mat'  Measurements=None  UNITS=SI  NominalPower=FullLoop.tiModules(4).Pn_fn  Winding1=FullLoop.tiModules(4).W1  Winding2=FullLoop.tiModules(4).W2  Winding3=[3.15e+05 1.2118e+09 4.0926e+05]  Saturation=FullLoop.tiModules(4).Sat  CoreLoss=TI_OCEM.Rm  BreakLoop=off  DiscreteSolver=Trapezoidal iterative  DataType=on  InitialFlux=0.0205600583592649  TransfoNumber=1
      settings: LibrarySourceBlock=sps_lib/Power Grid Elements/Saturable Transformer
  TI_005_F39_02 : spsSaturableTransformerLib/Saturable Transformer  ThreeWindings=off  Hysteresis=off  DataFile='hysteresis.mat'  Measurements=None  UNITS=SI  NominalPower=FullLoop.tiModules(5).Pn_fn  Winding1=FullLoop.tiModules(5).W1  Winding2=FullLoop.tiModules(5).W2  Winding3=[3.15e+05 1.2118e+09 4.0926e+05]  Saturation=FullLoop.tiModules(5).Sat  CoreLoss=TI_OCEM.Rm  BreakLoop=off  DiscreteSolver=Trapezoidal iterative  DataType=on  InitialFlux=0.0205600583592649  TransfoNumber=1
      settings: LibrarySourceBlock=sps_lib/Power Grid Elements/Saturable Transformer
  TI_006_F39_03 : spsSaturableTransformerLib/Saturable Transformer  ThreeWindings=off  Hysteresis=off  DataFile='hysteresis.mat'  Measurements=None  UNITS=SI  NominalPower=FullLoop.tiModules(6).Pn_fn  Winding1=FullLoop.tiModules(6).W1  Winding2=FullLoop.tiModules(6).W2  Winding3=[3.15e+05 1.2118e+09 4.0926e+05]  Saturation=FullLoop.tiModules(6).Sat  CoreLoss=TI_OCEM.Rm  BreakLoop=off  DiscreteSolver=Trapezoidal iterative  DataType=on  InitialFlux=0.0205600583592649  TransfoNumber=1
      settings: LibrarySourceBlock=sps_lib/Power Grid Elements/Saturable Transformer
  TI_007_F39_04 : spsSaturableTransformerLib/Saturable Transformer  ThreeWindings=off  Hysteresis=off  DataFile='hysteresis.mat'  Measurements=None  UNITS=SI  NominalPower=FullLoop.tiModules(7).Pn_fn  Winding1=FullLoop.tiModules(7).W1  Winding2=FullLoop.tiModules(7).W2  Winding3=[3.15e+05 1.2118e+09 4.0926e+05]  Saturation=FullLoop.tiModules(7).Sat  CoreLoss=TI_OCEM.Rm  BreakLoop=off  DiscreteSolver=Trapezoidal iterative  DataType=on  InitialFlux=0.0205600583592649  TransfoNumber=1
      settings: LibrarySourceBlock=sps_lib/Power Grid Elements/Saturable Transformer
  TI_008_F39_05 : spsSaturableTransformerLib/Saturable Transformer  ThreeWindings=off  Hysteresis=off  DataFile='hysteresis.mat'  Measurements=None  UNITS=SI  NominalPower=FullLoop.tiModules(8).Pn_fn  Winding1=FullLoop.tiModules(8).W1  Winding2=FullLoop.tiModules(8).W2  Winding3=[3.15e+05 1.2118e+09 4.0926e+05]  Saturation=FullLoop.tiModules(8).Sat  CoreLoss=TI_OCEM.Rm  BreakLoop=off  DiscreteSolver=Trapezoidal iterative  DataType=on  InitialFlux=0.0205600583592649  TransfoNumber=1
      settings: LibrarySourceBlock=sps_lib/Power Grid Elements/Saturable Transformer
  TI_009_F39_06 : spsSaturableTransformerLib/Saturable Transformer  ThreeWindings=off  Hysteresis=off  DataFile='hysteresis.mat'  Measurements=None  UNITS=SI  NominalPower=FullLoop.tiModules(9).Pn_fn  Winding1=FullLoop.tiModules(9).W1  Winding2=FullLoop.tiModules(9).W2  Winding3=[3.15e+05 1.2118e+09 4.0926e+05]  Saturation=FullLoop.tiModules(9).Sat  CoreLoss=TI_OCEM.Rm  BreakLoop=off  DiscreteSolver=Trapezoidal iterative  DataType=on  InitialFlux=0.0205600583592649  TransfoNumber=1
      settings: LibrarySourceBlock=sps_lib/Power Grid Elements/Saturable Transformer
  TI_010_F39_07 : spsSaturableTransformerLib/Saturable Transformer  ThreeWindings=off  Hysteresis=off  DataFile='hysteresis.mat'  Measurements=None  UNITS=SI  NominalPower=FullLoop.tiModules(10).Pn_fn  Winding1=FullLoop.tiModules(10).W1  Winding2=FullLoop.tiModules(10).W2  Winding3=[3.15e+05 1.2118e+09 4.0926e+05]  Saturation=FullLoop.tiModules(10).Sat  CoreLoss=TI_OCEM.Rm  BreakLoop=off  DiscreteSolver=Trapezoidal iterative  DataType=on  InitialFlux=0.0205600583592649  TransfoNumber=1
      settings: LibrarySourceBlock=sps_lib/Power Grid Elements/Saturable Transformer
  TI_011_F39_08 : spsSaturableTransformerLib/Saturable Transformer  ThreeWindings=off  Hysteresis=off  DataFile='hysteresis.mat'  Measurements=None  UNITS=SI  NominalPower=FullLoop.tiModules(11).Pn_fn  Winding1=FullLoop.tiModules(11).W1  Winding2=FullLoop.tiModules(11).W2  Winding3=[3.15e+05 1.2118e+09 4.0926e+05]  Saturation=FullLoop.tiModules(11).Sat  CoreLoss=TI_OCEM.Rm  BreakLoop=off  DiscreteSolver=Trapezoidal iterative  DataType=on  InitialFlux=0.0205600583592649  TransfoNumber=1
      settings: LibrarySourceBlock=sps_lib/Power Grid Elements/Saturable Transformer
  TI_012_F39_09 : spsSaturableTransformerLib/Saturable Transformer  ThreeWindings=off  Hysteresis=off  DataFile='hysteresis.mat'  Measurements=None  UNITS=SI  NominalPower=FullLoop.tiModules(12).Pn_fn  Winding1=FullLoop.tiModules(12).W1  Winding2=FullLoop.tiModules(12).W2  Winding3=[3.15e+05 1.2118e+09 4.0926e+05]  Saturation=FullLoop.tiModules(12).Sat  CoreLoss=TI_OCEM.Rm  BreakLoop=off  DiscreteSolver=Trapezoidal iterative  DataType=on  InitialFlux=0.0205600583592649  TransfoNumber=1
      settings: LibrarySourceBlock=sps_lib/Power Grid Elements/Saturable Transformer
  TI_013_F39_10 : spsSaturableTransformerLib/Saturable Transformer  ThreeWindings=off  Hysteresis=off  DataFile='hysteresis.mat'  Measurements=None  UNITS=SI  NominalPower=FullLoop.tiModules(13).Pn_fn  Winding1=FullLoop.tiModules(13).W1  Winding2=FullLoop.tiModules(13).W2  Winding3=[3.15e+05 1.2118e+09 4.0926e+05]  Saturation=FullLoop.tiModules(13).Sat  CoreLoss=TI_OCEM.Rm  BreakLoop=off  DiscreteSolver=Trapezoidal iterative  DataType=on  InitialFlux=0.0205600583592649  TransfoNumber=1
      settings: LibrarySourceBlock=sps_lib/Power Grid Elements/Saturable Transformer
  TI_014_F39_11 : spsSaturableTransformerLib/Saturable Transformer  ThreeWindings=off  Hysteresis=off  DataFile='hysteresis.mat'  Measurements=None  UNITS=SI  NominalPower=FullLoop.tiModules(14).Pn_fn  Winding1=FullLoop.tiModules(14).W1  Winding2=FullLoop.tiModules(14).W2  Winding3=[3.15e+05 1.2118e+09 4.0926e+05]  Saturation=FullLoop.tiModules(14).Sat  CoreLoss=TI_OCEM.Rm  BreakLoop=off  DiscreteSolver=Trapezoidal iterative  DataType=on  InitialFlux=0.0205600583592649  TransfoNumber=1
      settings: LibrarySourceBlock=sps_lib/Power Grid Elements/Saturable Transformer
  TI_015_F39_12 : spsSaturableTransformerLib/Saturable Transformer  ThreeWindings=off  Hysteresis=off  DataFile='hysteresis.mat'  Measurements=None  UNITS=SI  NominalPower=FullLoop.tiModules(15).Pn_fn  Winding1=FullLoop.tiModules(15).W1  Winding2=FullLoop.tiModules(15).W2  Winding3=[3.15e+05 1.2118e+09 4.0926e+05]  Saturation=FullLoop.tiModules(15).Sat  CoreLoss=TI_OCEM.Rm  BreakLoop=off  DiscreteSolver=Trapezoidal iterative  DataType=on  InitialFlux=0.0205600583592649  TransfoNumber=1
      settings: LibrarySourceBlock=sps_lib/Power Grid Elements/Saturable Transformer
  TI_016_F39_13 : spsSaturableTransformerLib/Saturable Transformer  ThreeWindings=off  Hysteresis=off  DataFile='hysteresis.mat'  Measurements=None  UNITS=SI  NominalPower=FullLoop.tiModules(16).Pn_fn  Winding1=FullLoop.tiModules(16).W1  Winding2=FullLoop.tiModules(16).W2  Winding3=[3.15e+05 1.2118e+09 4.0926e+05]  Saturation=FullLoop.tiModules(16).Sat  CoreLoss=TI_OCEM.Rm  BreakLoop=off  DiscreteSolver=Trapezoidal iterative  DataType=on  InitialFlux=0.0205600583592649  TransfoNumber=1
      settings: LibrarySourceBlock=sps_lib/Power Grid Elements/Saturable Transformer
  TI_017_F39_14 : spsSaturableTransformerLib/Saturable Transformer  ThreeWindings=off  Hysteresis=off  DataFile='hysteresis.mat'  Measurements=None  UNITS=SI  NominalPower=FullLoop.tiModules(17).Pn_fn  Winding1=FullLoop.tiModules(17).W1  Winding2=FullLoop.tiModules(17).W2  Winding3=[3.15e+05 1.2118e+09 4.0926e+05]  Saturation=FullLoop.tiModules(17).Sat  CoreLoss=TI_OCEM.Rm  BreakLoop=off  DiscreteSolver=Trapezoidal iterative  DataType=on  InitialFlux=0.0205600583592649  TransfoNumber=1
      settings: LibrarySourceBlock=sps_lib/Power Grid Elements/Saturable Transformer
  TI_018_F39_15 : spsSaturableTransformerLib/Saturable Transformer  ThreeWindings=off  Hysteresis=off  DataFile='hysteresis.mat'  Measurements=None  UNITS=SI  NominalPower=FullLoop.tiModules(18).Pn_fn  Winding1=FullLoop.tiModules(18).W1  Winding2=FullLoop.tiModules(18).W2  Winding3=[3.15e+05 1.2118e+09 4.0926e+05]  Saturation=FullLoop.tiModules(18).Sat  CoreLoss=TI_OCEM.Rm  BreakLoop=off  DiscreteSolver=Trapezoidal iterative  DataType=on  InitialFlux=0.0205600583592649  TransfoNumber=1
      settings: LibrarySourceBlock=sps_lib/Power Grid Elements/Saturable Transformer
  TI_019_F39_16 : spsSaturableTransformerLib/Saturable Transformer  ThreeWindings=off  Hysteresis=off  DataFile='hysteresis.mat'  Measurements=None  UNITS=SI  NominalPower=FullLoop.tiModules(19).Pn_fn  Winding1=FullLoop.tiModules(19).W1  Winding2=FullLoop.tiModules(19).W2  Winding3=[3.15e+05 1.2118e+09 4.0926e+05]  Saturation=FullLoop.tiModules(19).Sat  CoreLoss=TI_OCEM.Rm  BreakLoop=off  DiscreteSolver=Trapezoidal iterative  DataType=on  InitialFlux=0.0205600583592649  TransfoNumber=1
      settings: LibrarySourceBlock=sps_lib/Power Grid Elements/Saturable Transformer
  TI_020_F39_17 : spsSaturableTransformerLib/Saturable Transformer  ThreeWindings=off  Hysteresis=off  DataFile='hysteresis.mat'  Measurements=None  UNITS=SI  NominalPower=FullLoop.tiModules(20).Pn_fn  Winding1=FullLoop.tiModules(20).W1  Winding2=FullLoop.tiModules(20).W2  Winding3=[3.15e+05 1.2118e+09 4.0926e+05]  Saturation=FullLoop.tiModules(20).Sat  CoreLoss=TI_OCEM.Rm  BreakLoop=off  DiscreteSolver=Trapezoidal iterative  DataType=on  InitialFlux=0.0205600583592649  TransfoNumber=1
      settings: LibrarySourceBlock=sps_lib/Power Grid Elements/Saturable Transformer
  TI_021_F39_18 : spsSaturableTransformerLib/Saturable Transformer  ThreeWindings=off  Hysteresis=off  DataFile='hysteresis.mat'  Measurements=None  UNITS=SI  NominalPower=FullLoop.tiModules(21).Pn_fn  Winding1=FullLoop.tiModules(21).W1  Winding2=FullLoop.tiModules(21).W2  Winding3=[3.15e+05 1.2118e+09 4.0926e+05]  Saturation=FullLoop.tiModules(21).Sat  CoreLoss=TI_OCEM.Rm  BreakLoop=off  DiscreteSolver=Trapezoidal iterative  DataType=on  InitialFlux=0.0205600583592649  TransfoNumber=1
      settings: LibrarySourceBlock=sps_lib/Power Grid Elements/Saturable Transformer
  TI_022_F39_19 : spsSaturableTransformerLib/Saturable Transformer  ThreeWindings=off  Hysteresis=off  DataFile='hysteresis.mat'  Measurements=None  UNITS=SI  NominalPower=FullLoop.tiModules(22).Pn_fn  Winding1=FullLoop.tiModules(22).W1  Winding2=FullLoop.tiModules(22).W2  Winding3=[3.15e+05 1.2118e+09 4.0926e+05]  Saturation=FullLoop.tiModules(22).Sat  CoreLoss=TI_OCEM.Rm  BreakLoop=off  DiscreteSolver=Trapezoidal iterative  DataType=on  InitialFlux=0.0205600583592649  TransfoNumber=1
      settings: LibrarySourceBlock=sps_lib/Power Grid Elements/Saturable Transformer
  TI_023_F39_20 : spsSaturableTransformerLib/Saturable Transformer  ThreeWindings=off  Hysteresis=off  DataFile='hysteresis.mat'  Measurements=None  UNITS=SI  NominalPower=FullLoop.tiModules(23).Pn_fn  Winding1=FullLoop.tiModules(23).W1  Winding2=FullLoop.tiModules(23).W2  Winding3=[3.15e+05 1.2118e+09 4.0926e+05]  Saturation=FullLoop.tiModules(23).Sat  CoreLoss=TI_OCEM.Rm  BreakLoop=off  DiscreteSolver=Trapezoidal iterative  DataType=on  InitialFlux=0.0205600583592649  TransfoNumber=1
      settings: LibrarySourceBlock=sps_lib/Power Grid Elements/Saturable Transformer
  TI_024_F39_21 : spsSaturableTransformerLib/Saturable Transformer  ThreeWindings=off  Hysteresis=off  DataFile='hysteresis.mat'  Measurements=None  UNITS=SI  NominalPower=FullLoop.tiModules(24).Pn_fn  Winding1=FullLoop.tiModules(24).W1  Winding2=FullLoop.tiModules(24).W2  Winding3=[3.15e+05 1.2118e+09 4.0926e+05]  Saturation=FullLoop.tiModules(24).Sat  CoreLoss=TI_OCEM.Rm  BreakLoop=off  DiscreteSolver=Trapezoidal iterative  DataType=on  InitialFlux=0.0205600583592649  TransfoNumber=1
      settings: LibrarySourceBlock=sps_lib/Power Grid Elements/Saturable Transformer
  TI_025_F39_22 : spsSaturableTransformerLib/Saturable Transformer  ThreeWindings=off  Hysteresis=off  DataFile='hysteresis.mat'  Measurements=None  UNITS=SI  NominalPower=FullLoop.tiModules(25).Pn_fn  Winding1=FullLoop.tiModules(25).W1  Winding2=FullLoop.tiModules(25).W2  Winding3=[3.15e+05 1.2118e+09 4.0926e+05]  Saturation=FullLoop.tiModules(25).Sat  CoreLoss=TI_OCEM.Rm  BreakLoop=off  DiscreteSolver=Trapezoidal iterative  DataType=on  InitialFlux=0.0205600583592649  TransfoNumber=1
      settings: LibrarySourceBlock=sps_lib/Power Grid Elements/Saturable Transformer
  TI_026_F39_23 : spsSaturableTransformerLib/Saturable Transformer  ThreeWindings=off  Hysteresis=off  DataFile='hysteresis.mat'  Measurements=None  UNITS=SI  NominalPower=FullLoop.tiModules(26).Pn_fn  Winding1=FullLoop.tiModules(26).W1  Winding2=FullLoop.tiModules(26).W2  Winding3=[3.15e+05 1.2118e+09 4.0926e+05]  Saturation=FullLoop.tiModules(26).Sat  CoreLoss=TI_OCEM.Rm  BreakLoop=off  DiscreteSolver=Trapezoidal iterative  DataType=on  InitialFlux=0.0205600583592649  TransfoNumber=1
      settings: LibrarySourceBlock=sps_lib/Power Grid Elements/Saturable Transformer
  TI_027_F8_01 : spsSaturableTransformerLib/Saturable Transformer  ThreeWindings=off  Hysteresis=off  DataFile='hysteresis.mat'  Measurements=None  UNITS=SI  NominalPower=FullLoop.tiModules(27).Pn_fn  Winding1=FullLoop.tiModules(27).W1  Winding2=FullLoop.tiModules(27).W2  Winding3=[3.15e+05 1.2118e+09 4.0926e+05]  Saturation=FullLoop.tiModules(27).Sat  CoreLoss=TI_OCEM.Rm  BreakLoop=off  DiscreteSolver=Trapezoidal iterative  DataType=on  InitialFlux=0.0205600583592649  TransfoNumber=1
      settings: LibrarySourceBlock=sps_lib/Power Grid Elements/Saturable Transformer
  TI_028_F8_02 : spsSaturableTransformerLib/Saturable Transformer  ThreeWindings=off  Hysteresis=off  DataFile='hysteresis.mat'  Measurements=None  UNITS=SI  NominalPower=FullLoop.tiModules(28).Pn_fn  Winding1=FullLoop.tiModules(28).W1  Winding2=FullLoop.tiModules(28).W2  Winding3=[3.15e+05 1.2118e+09 4.0926e+05]  Saturation=FullLoop.tiModules(28).Sat  CoreLoss=TI_OCEM.Rm  BreakLoop=off  DiscreteSolver=Trapezoidal iterative  DataType=on  InitialFlux=0.0205600583592649  TransfoNumber=1
      settings: LibrarySourceBlock=sps_lib/Power Grid Elements/Saturable Transformer
  TI_029_F8_03 : spsSaturableTransformerLib/Saturable Transformer  ThreeWindings=off  Hysteresis=off  DataFile='hysteresis.mat'  Measurements=None  UNITS=SI  NominalPower=FullLoop.tiModules(29).Pn_fn  Winding1=FullLoop.tiModules(29).W1  Winding2=FullLoop.tiModules(29).W2  Winding3=[3.15e+05 1.2118e+09 4.0926e+05]  Saturation=FullLoop.tiModules(29).Sat  CoreLoss=TI_OCEM.Rm  BreakLoop=off  DiscreteSolver=Trapezoidal iterative  DataType=on  InitialFlux=0.0205600583592649  TransfoNumber=1
      settings: LibrarySourceBlock=sps_lib/Power Grid Elements/Saturable Transformer
  TI_030_F8_04 : spsSaturableTransformerLib/Saturable Transformer  ThreeWindings=off  Hysteresis=off  DataFile='hysteresis.mat'  Measurements=None  UNITS=SI  NominalPower=FullLoop.tiModules(30).Pn_fn  Winding1=FullLoop.tiModules(30).W1  Winding2=FullLoop.tiModules(30).W2  Winding3=[3.15e+05 1.2118e+09 4.0926e+05]  Saturation=FullLoop.tiModules(30).Sat  CoreLoss=TI_OCEM.Rm  BreakLoop=off  DiscreteSolver=Trapezoidal iterative  DataType=on  InitialFlux=0.0205600583592649  TransfoNumber=1
      settings: LibrarySourceBlock=sps_lib/Power Grid Elements/Saturable Transformer
  TI_031_F8_05 : spsSaturableTransformerLib/Saturable Transformer  ThreeWindings=off  Hysteresis=off  DataFile='hysteresis.mat'  Measurements=None  UNITS=SI  NominalPower=FullLoop.tiModules(31).Pn_fn  Winding1=FullLoop.tiModules(31).W1  Winding2=FullLoop.tiModules(31).W2  Winding3=[3.15e+05 1.2118e+09 4.0926e+05]  Saturation=FullLoop.tiModules(31).Sat  CoreLoss=TI_OCEM.Rm  BreakLoop=off  DiscreteSolver=Trapezoidal iterative  DataType=on  InitialFlux=0.0205600583592649  TransfoNumber=1
      settings: LibrarySourceBlock=sps_lib/Power Grid Elements/Saturable Transformer
  TI_032_F8_06 : spsSaturableTransformerLib/Saturable Transformer  ThreeWindings=off  Hysteresis=off  DataFile='hysteresis.mat'  Measurements=None  UNITS=SI  NominalPower=FullLoop.tiModules(32).Pn_fn  Winding1=FullLoop.tiModules(32).W1  Winding2=FullLoop.tiModules(32).W2  Winding3=[3.15e+05 1.2118e+09 4.0926e+05]  Saturation=FullLoop.tiModules(32).Sat  CoreLoss=TI_OCEM.Rm  BreakLoop=off  DiscreteSolver=Trapezoidal iterative  DataType=on  InitialFlux=0.0205600583592649  TransfoNumber=1
      settings: LibrarySourceBlock=sps_lib/Power Grid Elements/Saturable Transformer
  TI_033_F8_07 : spsSaturableTransformerLib/Saturable Transformer  ThreeWindings=off  Hysteresis=off  DataFile='hysteresis.mat'  Measurements=None  UNITS=SI  NominalPower=FullLoop.tiModules(33).Pn_fn  Winding1=FullLoop.tiModules(33).W1  Winding2=FullLoop.tiModules(33).W2  Winding3=[3.15e+05 1.2118e+09 4.0926e+05]  Saturation=FullLoop.tiModules(33).Sat  CoreLoss=TI_OCEM.Rm  BreakLoop=off  DiscreteSolver=Trapezoidal iterative  DataType=on  InitialFlux=0.0205600583592649  TransfoNumber=1
      settings: LibrarySourceBlock=sps_lib/Power Grid Elements/Saturable Transformer
  TI_034_F8_08 : spsSaturableTransformerLib/Saturable Transformer  ThreeWindings=off  Hysteresis=off  DataFile='hysteresis.mat'  Measurements=None  UNITS=SI  NominalPower=FullLoop.tiModules(34).Pn_fn  Winding1=FullLoop.tiModules(34).W1  Winding2=FullLoop.tiModules(34).W2  Winding3=[3.15e+05 1.2118e+09 4.0926e+05]  Saturation=FullLoop.tiModules(34).Sat  CoreLoss=TI_OCEM.Rm  BreakLoop=off  DiscreteSolver=Trapezoidal iterative  DataType=on  InitialFlux=0.0205600583592649  TransfoNumber=1
      settings: LibrarySourceBlock=sps_lib/Power Grid Elements/Saturable Transformer
  TI_035_F8_09 : spsSaturableTransformerLib/Saturable Transformer  ThreeWindings=off  Hysteresis=off  DataFile='hysteresis.mat'  Measurements=None  UNITS=SI  NominalPower=FullLoop.tiModules(35).Pn_fn  Winding1=FullLoop.tiModules(35).W1  Winding2=FullLoop.tiModules(35).W2  Winding3=[3.15e+05 1.2118e+09 4.0926e+05]  Saturation=FullLoop.tiModules(35).Sat  CoreLoss=TI_OCEM.Rm  BreakLoop=off  DiscreteSolver=Trapezoidal iterative  DataType=on  InitialFlux=0.0205600583592649  TransfoNumber=1
      settings: LibrarySourceBlock=sps_lib/Power Grid Elements/Saturable Transformer
  TI_036_F8_10 : spsSaturableTransformerLib/Saturable Transformer  ThreeWindings=off  Hysteresis=off  DataFile='hysteresis.mat'  Measurements=None  UNITS=SI  NominalPower=FullLoop.tiModules(36).Pn_fn  Winding1=FullLoop.tiModules(36).W1  Winding2=FullLoop.tiModules(36).W2  Winding3=[3.15e+05 1.2118e+09 4.0926e+05]  Saturation=FullLoop.tiModules(36).Sat  CoreLoss=TI_OCEM.Rm  BreakLoop=off  DiscreteSolver=Trapezoidal iterative  DataType=on  InitialFlux=0.0205600583592649  TransfoNumber=1
      settings: LibrarySourceBlock=sps_lib/Power Grid Elements/Saturable Transformer
  TI_037_F8_11 : spsSaturableTransformerLib/Saturable Transformer  ThreeWindings=off  Hysteresis=off  DataFile='hysteresis.mat'  Measurements=None  UNITS=SI  NominalPower=FullLoop.tiModules(37).Pn_fn  Winding1=FullLoop.tiModules(37).W1  Winding2=FullLoop.tiModules(37).W2  Winding3=[3.15e+05 1.2118e+09 4.0926e+05]  Saturation=FullLoop.tiModules(37).Sat  CoreLoss=TI_OCEM.Rm  BreakLoop=off  DiscreteSolver=Trapezoidal iterative  DataType=on  InitialFlux=0.0205600583592649  TransfoNumber=1
      settings: LibrarySourceBlock=sps_lib/Power Grid Elements/Saturable Transformer
  TI_038_F8_12 : spsSaturableTransformerLib/Saturable Transformer  ThreeWindings=off  Hysteresis=off  DataFile='hysteresis.mat'  Measurements=None  UNITS=SI  NominalPower=FullLoop.tiModules(38).Pn_fn  Winding1=FullLoop.tiModules(38).W1  Winding2=FullLoop.tiModules(38).W2  Winding3=[3.15e+05 1.2118e+09 4.0926e+05]  Saturation=FullLoop.tiModules(38).Sat  CoreLoss=TI_OCEM.Rm  BreakLoop=off  DiscreteSolver=Trapezoidal iterative  DataType=on  InitialFlux=0.0205600583592649  TransfoNumber=1
      settings: LibrarySourceBlock=sps_lib/Power Grid Elements/Saturable Transformer
  TI_039_F8_13 : spsSaturableTransformerLib/Saturable Transformer  ThreeWindings=off  Hysteresis=off  DataFile='hysteresis.mat'  Measurements=None  UNITS=SI  NominalPower=FullLoop.tiModules(39).Pn_fn  Winding1=FullLoop.tiModules(39).W1  Winding2=FullLoop.tiModules(39).W2  Winding3=[3.15e+05 1.2118e+09 4.0926e+05]  Saturation=FullLoop.tiModules(39).Sat  CoreLoss=TI_OCEM.Rm  BreakLoop=off  DiscreteSolver=Trapezoidal iterative  DataType=on  InitialFlux=0.0205600583592649  TransfoNumber=1
      settings: LibrarySourceBlock=sps_lib/Power Grid Elements/Saturable Transformer
  TI_040_F23_01 : spsSaturableTransformerLib/Saturable Transformer  ThreeWindings=off  Hysteresis=off  DataFile='hysteresis.mat'  Measurements=None  UNITS=SI  NominalPower=FullLoop.tiModules(40).Pn_fn  Winding1=FullLoop.tiModules(40).W1  Winding2=FullLoop.tiModules(40).W2  Winding3=[3.15e+05 1.2118e+09 4.0926e+05]  Saturation=FullLoop.tiModules(40).Sat  CoreLoss=TI_OCEM.Rm  BreakLoop=off  DiscreteSolver=Trapezoidal iterative  DataType=on  InitialFlux=0.0205600583592649  TransfoNumber=1
      settings: LibrarySourceBlock=sps_lib/Power Grid Elements/Saturable Transformer
  TI_041_F23_02 : spsSaturableTransformerLib/Saturable Transformer  ThreeWindings=off  Hysteresis=off  DataFile='hysteresis.mat'  Measurements=None  UNITS=SI  NominalPower=FullLoop.tiModules(41).Pn_fn  Winding1=FullLoop.tiModules(41).W1  Winding2=FullLoop.tiModules(41).W2  Winding3=[3.15e+05 1.2118e+09 4.0926e+05]  Saturation=FullLoop.tiModules(41).Sat  CoreLoss=TI_OCEM.Rm  BreakLoop=off  DiscreteSolver=Trapezoidal iterative  DataType=on  InitialFlux=0.0205600583592649  TransfoNumber=1
      settings: LibrarySourceBlock=sps_lib/Power Grid Elements/Saturable Transformer
  TI_042_F23_03 : spsSaturableTransformerLib/Saturable Transformer  ThreeWindings=off  Hysteresis=off  DataFile='hysteresis.mat'  Measurements=None  UNITS=SI  NominalPower=FullLoop.tiModules(42).Pn_fn  Winding1=FullLoop.tiModules(42).W1  Winding2=FullLoop.tiModules(42).W2  Winding3=[3.15e+05 1.2118e+09 4.0926e+05]  Saturation=FullLoop.tiModules(42).Sat  CoreLoss=TI_OCEM.Rm  BreakLoop=off  DiscreteSolver=Trapezoidal iterative  DataType=on  InitialFlux=0.0205600583592649  TransfoNumber=1
      settings: LibrarySourceBlock=sps_lib/Power Grid Elements/Saturable Transformer
  TI_043_F23_04 : spsSaturableTransformerLib/Saturable Transformer  ThreeWindings=off  Hysteresis=off  DataFile='hysteresis.mat'  Measurements=None  UNITS=SI  NominalPower=FullLoop.tiModules(43).Pn_fn  Winding1=FullLoop.tiModules(43).W1  Winding2=FullLoop.tiModules(43).W2  Winding3=[3.15e+05 1.2118e+09 4.0926e+05]  Saturation=FullLoop.tiModules(43).Sat  CoreLoss=TI_OCEM.Rm  BreakLoop=off  DiscreteSolver=Trapezoidal iterative  DataType=on  InitialFlux=0.0205600583592649  TransfoNumber=1
      settings: LibrarySourceBlock=sps_lib/Power Grid Elements/Saturable Transformer
  TI_044_F23_05 : spsSaturableTransformerLib/Saturable Transformer  ThreeWindings=off  Hysteresis=off  DataFile='hysteresis.mat'  Measurements=None  UNITS=SI  NominalPower=FullLoop.tiModules(44).Pn_fn  Winding1=FullLoop.tiModules(44).W1  Winding2=FullLoop.tiModules(44).W2  Winding3=[3.15e+05 1.2118e+09 4.0926e+05]  Saturation=FullLoop.tiModules(44).Sat  CoreLoss=TI_OCEM.Rm  BreakLoop=off  DiscreteSolver=Trapezoidal iterative  DataType=on  InitialFlux=0.0205600583592649  TransfoNumber=1
      settings: LibrarySourceBlock=sps_lib/Power Grid Elements/Saturable Transformer
  TI_045_F23_06 : spsSaturableTransformerLib/Saturable Transformer  ThreeWindings=off  Hysteresis=off  DataFile='hysteresis.mat'  Measurements=None  UNITS=SI  NominalPower=FullLoop.tiModules(45).Pn_fn  Winding1=FullLoop.tiModules(45).W1  Winding2=FullLoop.tiModules(45).W2  Winding3=[3.15e+05 1.2118e+09 4.0926e+05]  Saturation=FullLoop.tiModules(45).Sat  CoreLoss=TI_OCEM.Rm  BreakLoop=off  DiscreteSolver=Trapezoidal iterative  DataType=on  InitialFlux=0.0205600583592649  TransfoNumber=1
      settings: LibrarySourceBlock=sps_lib/Power Grid Elements/Saturable Transformer
  TI_046_F22_01 : spsSaturableTransformerLib/Saturable Transformer  ThreeWindings=off  Hysteresis=off  DataFile='hysteresis.mat'  Measurements=None  UNITS=SI  NominalPower=FullLoop.tiModules(46).Pn_fn  Winding1=FullLoop.tiModules(46).W1  Winding2=FullLoop.tiModules(46).W2  Winding3=[3.15e+05 1.2118e+09 4.0926e+05]  Saturation=FullLoop.tiModules(46).Sat  CoreLoss=TI_OCEM.Rm  BreakLoop=off  DiscreteSolver=Trapezoidal iterative  DataType=on  InitialFlux=0.0205600583592649  TransfoNumber=1
      settings: LibrarySourceBlock=sps_lib/Power Grid Elements/Saturable Transformer
  TI_047_F22_02 : spsSaturableTransformerLib/Saturable Transformer  ThreeWindings=off  Hysteresis=off  DataFile='hysteresis.mat'  Measurements=None  UNITS=SI  NominalPower=FullLoop.tiModules(47).Pn_fn  Winding1=FullLoop.tiModules(47).W1  Winding2=FullLoop.tiModules(47).W2  Winding3=[3.15e+05 1.2118e+09 4.0926e+05]  Saturation=FullLoop.tiModules(47).Sat  CoreLoss=TI_OCEM.Rm  BreakLoop=off  DiscreteSolver=Trapezoidal iterative  DataType=on  InitialFlux=0.0205600583592649  TransfoNumber=1
      settings: LibrarySourceBlock=sps_lib/Power Grid Elements/Saturable Transformer
  TI_048_WINDCONE_01_TI_1 : spsSaturableTransformerLib/Saturable Transformer  ThreeWindings=off  Hysteresis=off  DataFile='hysteresis.mat'  Measurements=None  UNITS=SI  NominalPower=FullLoop.tiModules(48).Pn_fn  Winding1=FullLoop.tiModules(48).W1  Winding2=FullLoop.tiModules(48).W2  Winding3=[3.15e+05 1.2118e+09 4.0926e+05]  Saturation=FullLoop.tiModules(48).Sat  CoreLoss=TI_OCEM.Rm  BreakLoop=off  DiscreteSolver=Trapezoidal iterative  DataType=on  InitialFlux=0.0205600583592649  TransfoNumber=1
      settings: LibrarySourceBlock=sps_lib/Power Grid Elements/Saturable Transformer
  TI_049_WINDCONE_01_TI_2 : spsSaturableTransformerLib/Saturable Transformer  ThreeWindings=off  Hysteresis=off  DataFile='hysteresis.mat'  Measurements=None  UNITS=SI  NominalPower=FullLoop.tiModules(49).Pn_fn  Winding1=FullLoop.tiModules(49).W1  Winding2=FullLoop.tiModules(49).W2  Winding3=[3.15e+05 1.2118e+09 4.0926e+05]  Saturation=FullLoop.tiModules(49).Sat  CoreLoss=TI_OCEM.Rm  BreakLoop=off  DiscreteSolver=Trapezoidal iterative  DataType=on  InitialFlux=0.0205600583592649  TransfoNumber=1
      settings: LibrarySourceBlock=sps_lib/Power Grid Elements/Saturable Transformer
  TI_050_WINDCONE_02_TI_1 : spsSaturableTransformerLib/Saturable Transformer  ThreeWindings=off  Hysteresis=off  DataFile='hysteresis.mat'  Measurements=None  UNITS=SI  NominalPower=FullLoop.tiModules(50).Pn_fn  Winding1=FullLoop.tiModules(50).W1  Winding2=FullLoop.tiModules(50).W2  Winding3=[3.15e+05 1.2118e+09 4.0926e+05]  Saturation=FullLoop.tiModules(50).Sat  CoreLoss=TI_OCEM.Rm  BreakLoop=off  DiscreteSolver=Trapezoidal iterative  DataType=on  InitialFlux=0.0205600583592649  TransfoNumber=1
      settings: LibrarySourceBlock=sps_lib/Power Grid Elements/Saturable Transformer
  TI_051_WINDCONE_02_TI_2 : spsSaturableTransformerLib/Saturable Transformer  ThreeWindings=off  Hysteresis=off  DataFile='hysteresis.mat'  Measurements=None  UNITS=SI  NominalPower=FullLoop.tiModules(51).Pn_fn  Winding1=FullLoop.tiModules(51).W1  Winding2=FullLoop.tiModules(51).W2  Winding3=[3.15e+05 1.2118e+09 4.0926e+05]  Saturation=FullLoop.tiModules(51).Sat  CoreLoss=TI_OCEM.Rm  BreakLoop=off  DiscreteSolver=Trapezoidal iterative  DataType=on  InitialFlux=0.0205600583592649  TransfoNumber=1
      settings: LibrarySourceBlock=sps_lib/Power Grid Elements/Saturable Transformer
  ToWorkspace_I_MEAS_001 : ToWorkspace  VariableName=FullLoop_I_MEAS_001  SaveFormat=Timeseries  SampleTime=-1
  ToWorkspace_I_MEAS_010 : ToWorkspace  VariableName=FullLoop_I_MEAS_010  SaveFormat=Timeseries  SampleTime=-1
  ToWorkspace_I_MEAS_020 : ToWorkspace  VariableName=FullLoop_I_MEAS_020  SaveFormat=Timeseries  SampleTime=-1
  ToWorkspace_I_MEAS_030 : ToWorkspace  VariableName=FullLoop_I_MEAS_030  SaveFormat=Timeseries  SampleTime=-1
  ToWorkspace_I_MEAS_040 : ToWorkspace  VariableName=FullLoop_I_MEAS_040  SaveFormat=Timeseries  SampleTime=-1
  ToWorkspace_I_MEAS_050 : ToWorkspace  VariableName=FullLoop_I_MEAS_050  SaveFormat=Timeseries  SampleTime=-1
  ToWorkspace_I_MEAS_051 : ToWorkspace  VariableName=FullLoop_I_MEAS_051  SaveFormat=Timeseries  SampleTime=-1
  ToWorkspace_i_RCC : ToWorkspace  VariableName=i_RCC  SaveFormat=Timeseries  SampleTime=-1
  ToWorkspace_u_RCC : ToWorkspace  VariableName=u_RCC  SaveFormat=Timeseries  SampleTime=-1
  powergui : spspowerguiLib/powergui  Priority=1  SimulationMode=Discrete  SampleTime=DIAM4100.powergui.Ts_s  frequency=DIAM4100.grid.f_Hz  Iterations=50  frequencyindice=DIAM4100.grid.f_Hz  Pbase=100e6  ErrMax=1e-4  UnitsV=kV  UnitsW=MW  buscounter=0  FunctionMessages=off  echomessages=off  EnableUseOfTLC=off  CurrentSourceSwitches=off  DisableSnubberDevices=off  DisableRonSwitches=off  DisableVfSwitches=off  DisplayEquations=off  AutomaticDiscreteSolvers=off  SolverType=Tustin/Backward Euler (TBE)  Interpol=off  ExternalGateDelay=off  methode=off  Ts=100  x0status=blocks  SPID=on  SwTol=0  HookPort=off  NonlinearTolerance=1e-4  nMaxIteration=100  ContinueOnMaxIteration=off  RestoreLinks=warning  ResistiveCurrentMeasurement=off  Frange=[0:2:500]  Ylog=off  Xlog=on  ShowGrid=off  save=off  variable=ZData  structure=0  ZoomFFT=off  StartTime=0.0  cycles=1  DisplayStyle=1  fundamental=DIAM4100.grid.f_Hz  FreqAxis=off  MaxFrequency=1000  frequencyindicesteady=1  RmsSteady=1  display=off
  wires:
  I_MEAS_001/1 -> ToWorkspace_I_MEAS_001/1
  I_MEAS_010/1 -> ToWorkspace_I_MEAS_010/1
  I_MEAS_020/1 -> ToWorkspace_I_MEAS_020/1
  I_MEAS_030/1 -> ToWorkspace_I_MEAS_030/1
  I_MEAS_040/1 -> ToWorkspace_I_MEAS_040/1
  I_MEAS_050/1 -> ToWorkspace_I_MEAS_050/1
  I_MEAS_051/1 -> ToWorkspace_I_MEAS_051/1
  RCC Voltage Measurement/1 -> ToWorkspace_u_RCC/1
  Current Measurement/1 -> ToWorkspace_i_RCC/1
  connections:
  Cable_001/RConn1 -- I_MEAS_001/LConn1
  I_MEAS_001/RConn1 -- TI_001_F65_01/LConn1
  TI_001_F65_01/RConn1 -- LOAD_001_F65_01/LConn1
  LOAD_001_F65_01/RConn1 -- TI_001_F65_01/RConn2
  TI_001_F65_01/LConn2 -- Cable_002/LConn1
  Cable_002/RConn1 -- TI_002_F65_02/LConn1
  TI_002_F65_02/RConn1 -- LOAD_002_F65_02/LConn1
  LOAD_002_F65_02/RConn1 -- TI_002_F65_02/RConn2
  TI_002_F65_02/LConn2 -- Cable_003/LConn1
  Cable_003/RConn1 -- TI_003_F65_03/LConn1
  TI_003_F65_03/RConn1 -- LOAD_003_F65_03/LConn1
  LOAD_003_F65_03/RConn1 -- TI_003_F65_03/RConn2
  TI_003_F65_03/LConn2 -- Cable_004/LConn1
  Cable_004/RConn1 -- TI_004_F39_01/LConn1
  TI_004_F39_01/RConn1 -- LOAD_004_F39_01/LConn1
  LOAD_004_F39_01/RConn1 -- TI_004_F39_01/RConn2
  TI_004_F39_01/LConn2 -- Cable_005/LConn1
  Cable_005/RConn1 -- TI_005_F39_02/LConn1
  TI_005_F39_02/RConn1 -- LOAD_005_F39_02/LConn1
  LOAD_005_F39_02/RConn1 -- TI_005_F39_02/RConn2
  TI_005_F39_02/LConn2 -- Cable_006/LConn1
  Cable_006/RConn1 -- TI_006_F39_03/LConn1
  TI_006_F39_03/RConn1 -- LOAD_006_F39_03/LConn1
  LOAD_006_F39_03/RConn1 -- TI_006_F39_03/RConn2
  TI_006_F39_03/LConn2 -- Cable_007/LConn1
  Cable_007/RConn1 -- TI_007_F39_04/LConn1
  TI_007_F39_04/RConn1 -- LOAD_007_F39_04/LConn1
  LOAD_007_F39_04/RConn1 -- TI_007_F39_04/RConn2
  TI_007_F39_04/LConn2 -- Cable_008/LConn1
  Cable_008/RConn1 -- TI_008_F39_05/LConn1
  TI_008_F39_05/RConn1 -- LOAD_008_F39_05/LConn1
  LOAD_008_F39_05/RConn1 -- TI_008_F39_05/RConn2
  TI_008_F39_05/LConn2 -- Cable_009/LConn1
  Cable_009/RConn1 -- TI_009_F39_06/LConn1
  TI_009_F39_06/RConn1 -- LOAD_009_F39_06/LConn1
  LOAD_009_F39_06/RConn1 -- TI_009_F39_06/RConn2
  TI_009_F39_06/LConn2 -- Cable_010/LConn1
  Cable_010/RConn1 -- I_MEAS_010/LConn1
  I_MEAS_010/RConn1 -- TI_010_F39_07/LConn1
  TI_010_F39_07/RConn1 -- LOAD_010_F39_07/LConn1
  LOAD_010_F39_07/RConn1 -- TI_010_F39_07/RConn2
  Cable_011/RConn1 -- TI_011_F39_08/LConn1
  TI_011_F39_08/RConn1 -- LOAD_011_F39_08/LConn1
  LOAD_011_F39_08/RConn1 -- TI_011_F39_08/RConn2
  TI_011_F39_08/LConn2 -- Cable_012/LConn1
  Cable_012/RConn1 -- TI_012_F39_09/LConn1
  TI_012_F39_09/RConn1 -- LOAD_012_F39_09/LConn1
  LOAD_012_F39_09/RConn1 -- TI_012_F39_09/RConn2
  TI_012_F39_09/LConn2 -- Cable_013/LConn1
  Cable_013/RConn1 -- TI_013_F39_10/LConn1
  TI_013_F39_10/RConn1 -- LOAD_013_F39_10/LConn1
  LOAD_013_F39_10/RConn1 -- TI_013_F39_10/RConn2
  TI_013_F39_10/LConn2 -- Cable_014/LConn1
  Cable_014/RConn1 -- TI_014_F39_11/LConn1
  TI_014_F39_11/RConn1 -- LOAD_014_F39_11/LConn1
  LOAD_014_F39_11/RConn1 -- TI_014_F39_11/RConn2
  TI_014_F39_11/LConn2 -- Cable_015/LConn1
  Cable_015/RConn1 -- TI_015_F39_12/LConn1
  TI_015_F39_12/RConn1 -- LOAD_015_F39_12/LConn1
  LOAD_015_F39_12/RConn1 -- TI_015_F39_12/RConn2
  TI_015_F39_12/LConn2 -- Cable_016/LConn1
  Cable_016/RConn1 -- TI_016_F39_13/LConn1
  TI_016_F39_13/RConn1 -- LOAD_016_F39_13/LConn1
  LOAD_016_F39_13/RConn1 -- TI_016_F39_13/RConn2
  TI_016_F39_13/LConn2 -- Cable_017/LConn1
  Cable_017/RConn1 -- TI_017_F39_14/LConn1
  TI_017_F39_14/RConn1 -- LOAD_017_F39_14/LConn1
  LOAD_017_F39_14/RConn1 -- TI_017_F39_14/RConn2
  TI_017_F39_14/LConn2 -- Cable_018/LConn1
  Cable_018/RConn1 -- TI_018_F39_15/LConn1
  TI_018_F39_15/RConn1 -- LOAD_018_F39_15/LConn1
  LOAD_018_F39_15/RConn1 -- TI_018_F39_15/RConn2
  TI_018_F39_15/LConn2 -- Cable_019/LConn1
  Cable_019/RConn1 -- TI_019_F39_16/LConn1
  TI_019_F39_16/RConn1 -- LOAD_019_F39_16/LConn1
  LOAD_019_F39_16/RConn1 -- TI_019_F39_16/RConn2
  TI_019_F39_16/LConn2 -- Cable_020/LConn1
  Cable_020/RConn1 -- I_MEAS_020/LConn1
  I_MEAS_020/RConn1 -- TI_020_F39_17/LConn1
  TI_020_F39_17/RConn1 -- LOAD_020_F39_17/LConn1
  LOAD_020_F39_17/RConn1 -- TI_020_F39_17/RConn2
  TI_020_F39_17/LConn2 -- Cable_021/LConn1
  Cable_021/RConn1 -- TI_021_F39_18/LConn1
  TI_021_F39_18/RConn1 -- LOAD_021_F39_18/LConn1
  LOAD_021_F39_18/RConn1 -- TI_021_F39_18/RConn2
  TI_021_F39_18/LConn2 -- Cable_022/LConn1
  Cable_022/RConn1 -- TI_022_F39_19/LConn1
  TI_022_F39_19/RConn1 -- LOAD_022_F39_19/LConn1
  LOAD_022_F39_19/RConn1 -- TI_022_F39_19/RConn2
  TI_022_F39_19/LConn2 -- Cable_023/LConn1
  Cable_023/RConn1 -- TI_023_F39_20/LConn1
  TI_023_F39_20/RConn1 -- LOAD_023_F39_20/LConn1
  LOAD_023_F39_20/RConn1 -- TI_023_F39_20/RConn2
  TI_023_F39_20/LConn2 -- Cable_024/LConn1
  Cable_024/RConn1 -- TI_024_F39_21/LConn1
  TI_024_F39_21/RConn1 -- LOAD_024_F39_21/LConn1
  LOAD_024_F39_21/RConn1 -- TI_024_F39_21/RConn2
  TI_024_F39_21/LConn2 -- Cable_025/LConn1
  Cable_025/RConn1 -- TI_025_F39_22/LConn1
  TI_025_F39_22/RConn1 -- LOAD_025_F39_22/LConn1
  LOAD_025_F39_22/RConn1 -- TI_025_F39_22/RConn2
  TI_025_F39_22/LConn2 -- Cable_026/LConn1
  Cable_026/RConn1 -- TI_026_F39_23/LConn1
  TI_026_F39_23/RConn1 -- LOAD_026_F39_23/LConn1
  LOAD_026_F39_23/RConn1 -- TI_026_F39_23/RConn2
  TI_026_F39_23/LConn2 -- Cable_027/LConn1
  Cable_027/RConn1 -- TI_027_F8_01/LConn1
  TI_027_F8_01/RConn1 -- LOAD_027_F8_01/LConn1
  LOAD_027_F8_01/RConn1 -- TI_027_F8_01/RConn2
  TI_027_F8_01/LConn2 -- Cable_028/LConn1
  Cable_028/RConn1 -- TI_028_F8_02/LConn1
  TI_028_F8_02/RConn1 -- LOAD_028_F8_02/LConn1
  LOAD_028_F8_02/RConn1 -- TI_028_F8_02/RConn2
  TI_028_F8_02/LConn2 -- Cable_029/LConn1
  Cable_029/RConn1 -- TI_029_F8_03/LConn1
  TI_029_F8_03/RConn1 -- LOAD_029_F8_03/LConn1
  LOAD_029_F8_03/RConn1 -- TI_029_F8_03/RConn2
  TI_029_F8_03/LConn2 -- Cable_030/LConn1
  Cable_030/RConn1 -- I_MEAS_030/LConn1
  I_MEAS_030/RConn1 -- TI_030_F8_04/LConn1
  TI_030_F8_04/RConn1 -- LOAD_030_F8_04/LConn1
  LOAD_030_F8_04/RConn1 -- TI_030_F8_04/RConn2
  TI_030_F8_04/LConn2 -- Cable_031/LConn1
  Cable_031/RConn1 -- TI_031_F8_05/LConn1
  TI_031_F8_05/RConn1 -- LOAD_031_F8_05/LConn1
  LOAD_031_F8_05/RConn1 -- TI_031_F8_05/RConn2
  TI_031_F8_05/LConn2 -- Cable_032/LConn1
  Cable_032/RConn1 -- TI_032_F8_06/LConn1
  TI_032_F8_06/RConn1 -- LOAD_032_F8_06/LConn1
  LOAD_032_F8_06/RConn1 -- TI_032_F8_06/RConn2
  TI_032_F8_06/LConn2 -- Cable_033/LConn1
  Cable_033/RConn1 -- TI_033_F8_07/LConn1
  TI_033_F8_07/RConn1 -- LOAD_033_F8_07/LConn1
  LOAD_033_F8_07/RConn1 -- TI_033_F8_07/RConn2
  TI_033_F8_07/LConn2 -- Cable_034/LConn1
  Cable_034/RConn1 -- TI_034_F8_08/LConn1
  TI_034_F8_08/RConn1 -- LOAD_034_F8_08/LConn1
  LOAD_034_F8_08/RConn1 -- TI_034_F8_08/RConn2
  TI_034_F8_08/LConn2 -- Cable_035/LConn1
  Cable_035/RConn1 -- TI_035_F8_09/LConn1
  TI_035_F8_09/RConn1 -- LOAD_035_F8_09/LConn1
  LOAD_035_F8_09/RConn1 -- TI_035_F8_09/RConn2
  TI_035_F8_09/LConn2 -- Cable_036/LConn1
  Cable_036/RConn1 -- TI_036_F8_10/LConn1
  TI_036_F8_10/RConn1 -- LOAD_036_F8_10/LConn1
  LOAD_036_F8_10/RConn1 -- TI_036_F8_10/RConn2
  TI_036_F8_10/LConn2 -- Cable_037/LConn1
  Cable_037/RConn1 -- TI_037_F8_11/LConn1
  TI_037_F8_11/RConn1 -- LOAD_037_F8_11/LConn1
  LOAD_037_F8_11/RConn1 -- TI_037_F8_11/RConn2
  TI_037_F8_11/LConn2 -- Cable_038/LConn1
  Cable_038/RConn1 -- TI_038_F8_12/LConn1
  TI_038_F8_12/RConn1 -- LOAD_038_F8_12/LConn1
  LOAD_038_F8_12/RConn1 -- TI_038_F8_12/RConn2
  TI_038_F8_12/LConn2 -- Cable_039/LConn1
  Cable_039/RConn1 -- TI_039_F8_13/LConn1
  TI_039_F8_13/RConn1 -- LOAD_039_F8_13/LConn1
  LOAD_039_F8_13/RConn1 -- TI_039_F8_13/RConn2
  TI_039_F8_13/LConn2 -- Cable_040/LConn1
  Cable_040/RConn1 -- I_MEAS_040/LConn1
  I_MEAS_040/RConn1 -- TI_040_F23_01/LConn1
  TI_040_F23_01/RConn1 -- LOAD_040_F23_01/LConn1
  LOAD_040_F23_01/RConn1 -- TI_040_F23_01/RConn2
  TI_040_F23_01/LConn2 -- Cable_041/LConn1
  Cable_041/RConn1 -- TI_041_F23_02/LConn1
  TI_041_F23_02/RConn1 -- LOAD_041_F23_02/LConn1
  LOAD_041_F23_02/RConn1 -- TI_041_F23_02/RConn2
  TI_041_F23_02/LConn2 -- Cable_042/LConn1
  Cable_042/RConn1 -- TI_042_F23_03/LConn1
  TI_042_F23_03/RConn1 -- LOAD_042_F23_03/LConn1
  LOAD_042_F23_03/RConn1 -- TI_042_F23_03/RConn2
  TI_042_F23_03/LConn2 -- Cable_043/LConn1
  Cable_043/RConn1 -- TI_043_F23_04/LConn1
  TI_043_F23_04/RConn1 -- LOAD_043_F23_04/LConn1
  LOAD_043_F23_04/RConn1 -- TI_043_F23_04/RConn2
  TI_043_F23_04/LConn2 -- Cable_044/LConn1
  Cable_044/RConn1 -- TI_044_F23_05/LConn1
  TI_044_F23_05/RConn1 -- LOAD_044_F23_05/LConn1
  LOAD_044_F23_05/RConn1 -- TI_044_F23_05/RConn2
  TI_044_F23_05/LConn2 -- Cable_045/LConn1
  Cable_045/RConn1 -- TI_045_F23_06/LConn1
  TI_045_F23_06/RConn1 -- LOAD_045_F23_06/LConn1
  LOAD_045_F23_06/RConn1 -- TI_045_F23_06/RConn2
  TI_045_F23_06/LConn2 -- Cable_046/LConn1
  Cable_046/RConn1 -- TI_046_F22_01/LConn1
  TI_046_F22_01/RConn1 -- LOAD_046_F22_01/LConn1
  LOAD_046_F22_01/RConn1 -- TI_046_F22_01/RConn2
  TI_046_F22_01/LConn2 -- Cable_047/LConn1
  Cable_047/RConn1 -- TI_047_F22_02/LConn1
  TI_047_F22_02/RConn1 -- LOAD_047_F22_02/LConn1
  LOAD_047_F22_02/RConn1 -- TI_047_F22_02/RConn2
  TI_047_F22_02/LConn2 -- Cable_048/LConn1
  Cable_048/RConn1 -- TI_048_WINDCONE_01_TI_1/LConn1
  TI_048_WINDCONE_01_TI_1/RConn1 -- LOAD_048_WINDCONE_01_TI_1/LConn1
  LOAD_048_WINDCONE_01_TI_1/RConn1 -- TI_048_WINDCONE_01_TI_1/RConn2
  TI_048_WINDCONE_01_TI_1/LConn2 -- TI_049_WINDCONE_01_TI_2/LConn1
  TI_049_WINDCONE_01_TI_2/RConn1 -- LOAD_049_WINDCONE_01_TI_2/LConn1
  LOAD_049_WINDCONE_01_TI_2/RConn1 -- TI_049_WINDCONE_01_TI_2/RConn2
  TI_049_WINDCONE_01_TI_2/LConn2 -- Cable_049/LConn1
  Cable_049/RConn1 -- I_MEAS_050/LConn1
  I_MEAS_050/RConn1 -- TI_050_WINDCONE_02_TI_1/LConn1
  TI_050_WINDCONE_02_TI_1/RConn1 -- LOAD_050_WINDCONE_02_TI_1/LConn1
  LOAD_050_WINDCONE_02_TI_1/RConn1 -- TI_050_WINDCONE_02_TI_1/RConn2
  TI_050_WINDCONE_02_TI_1/LConn2 -- I_MEAS_051/LConn1
  I_MEAS_051/RConn1 -- TI_051_WINDCONE_02_TI_2/LConn1
  TI_051_WINDCONE_02_TI_2/RConn1 -- LOAD_051_WINDCONE_02_TI_2/LConn1
  LOAD_051_WINDCONE_02_TI_2/RConn1 -- TI_051_WINDCONE_02_TI_2/RConn2
  TI_051_WINDCONE_02_TI_2/LConn2 -- Cable_050/LConn1
  TI_010_F39_07/LConn2 -- Cable_011/LConn1
  Cable_050/RConn1 -- Diam4100_CCR/RConn2 -- RCC Voltage Measurement/LConn2
  Current Measurement/LConn1 -- RCC Voltage Measurement/LConn1 -- Diam4100_CCR/RConn1
  Current Measurement/RConn1 -- Cable_001/LConn1
